simulink model "DualStreamSSR"  (R2021a)
(part 4 of 5)

      KernelAllAttrs=|
      | s[12;12;9;9;19;14;21;23;24;21;12;24;26;26;26;27;28;9;21;23;23;23;24;25;14;19;19;29]@FunctionNameDeclFileNamePortNamesPortTypesPortSerializedTypesPortDirectionsPortWindowSizeEnablesPortWindowMarginEnablesPortSynchronicityEnablesPortSignalSizeEnablesFunctionDeclFunctionTemplateSpecKindFunctionTemplateParamNamesFunctionTemplateParamKindsFunctionTemplateParamTypesFunctionTemplateParamValuesFunctionTemplateParamEnablesClassDeclClassTemplateSpecKindClassTemplateParamNamesClassTemplateParamKindsClassTemplateParamTypesClassTemplateParamValuesClassTemplateParamEnablesClassCtorDeclsClassCtorParamNamesClassCtorParamTypesClassCtorParamSerializedTypes[1 1]@C[28 1]@t6@filtert42@../../../aie/aie_kernels/FirDoubleStream.hC[4 1]@t4@sin1t4@sin2t3@cint4@coutC[4 1]@t30@input_stream_cint16 * restrictt30@input_stream_cint16 * restrictt26@input_stream< cacc48_t > *t27@output_stream< cacc48_t > *C[4 1]@t37@{Q2{P{Tinput_stream{1{t{Scint16}}}}}}t37@{Q2{P{Tinput_stream{1{t{Scint16}}}}}}t35@{P{Tinput_stream{1{t{Scacc48_t}}}}}t36@{P{Toutput_stream{1{t{Scacc48_t}}}}}C[4 1]@t5@inputt5@inputt5@inputt6@outputC[4 1]@l0@l0@l0@l0@C[4 1]@l0@l0@l0@l0@C[4 1]@l0@l0@l0@l0@C[4 1]@l0@l0@l0@l1@t281@namespace DoubleStream {
      | template < int NSamples, int ShiftAcc, bool DiscardSample, bool SwapRead > 
      | void FIR_MultiKernel_cincout::
      | filter(input_stream_cint16 * restrict sin1, input_stream_cint16 * restrict sin2, input_stream< cacc48_t > * cin, output_stream< cacc48_t > * cout);
      | }t4@nonee[0 1]@e[0 1]@e[0 1]@e[0 1]@e[0 1]@t132@namespace DoubleStream {
      | template < int NSamples, int ShiftAcc, bool DiscardSample, bool SwapRead > class FIR_MultiKernel_cincout;
      | }t8@implicitC[4 1]@t8@NSamplest8@ShiftAcct13@DiscardSamplet8@SwapReadC[4 1]@t7@nontypet7@nontypet7@nontypet7@nontypeC[4 1]@t3@intt3@intt4@boolt4@boolC[4 1]@nnnnC[4 1]@l1@l1@l1@l1@C[1 1]@t54@FIR_MultiKernel_cincout(cint16 const ( & taps ) [ 4 ])C[1 1]@C[1 1]@t4@tapsC[1 1]@C[1 1]@t23@cint16 const ( &) [ 4 ]C[1 1]@C[1 1]@t20@{R{Q1{C{Scint16}4}}}
      FunctionDecl=|
      | namespace DoubleStream {
      | template < int NSamples, int ShiftAcc, bool DiscardSample, bool SwapRead > 
      | void FIR_MultiKernel_cincout::
      | filter(input_stream_cint16 * restrict sin1, input_stream_cint16 * restrict sin2, input_stream< cacc48_t > * cin, output_stream< cacc48_t > * cout);
      | }
      ClassDeclTypeOptions=|
      | C[1 1]@t132@namespace DoubleStream {
      | template < int NSamples, int ShiftAcc, bool DiscardSample, bool SwapRead > class FIR_MultiKernel_cincout;
      | }
      ClassDecl=|
      | namespace DoubleStream {
      | template < int NSamples, int ShiftAcc, bool DiscardSample, bool SwapRead > class FIR_MultiKernel_cincout;
      | }
  filter53 : aieBasic/AIE Class Kernel  KernelAllAttrs=|  PortNames={'sin1'; 'sin2'; 'cin'; 'cout'}  PortSerializedTypes={'{Q2{P{Tinput_stream{1{t{Scint16}}}}}}'; '{Q2{P{Tinput_stream{1{t{Scint16}}}}}}'; '{P{Tinput_stream{1{t{Scacc48_t}}}}}'; '{P{Toutput_stream{1{t{Scacc48_t}}}}}'}  PortWindowSizes={0.000000000000000000e+00; 0.000000000000000000e+00; 0.000000000000000000e+00; 0.000000000000000000e+00}  PortWindowMargins={0.000000000000000000e+00; 0.000000000000000000e+00; 0.000000000000000000e+00; 0.000000000000000000e+00}  PortSynchronicities={'auto'; 'auto'; 'auto'; 'auto'}  PortSignalSizes={0.000000000000000000e+00; 0.000000000000000000e+00; 0.000000000000000000e+00; 8.000000000000000000e+00}  ClassTemplateSpecKind=implicit  ClassTemplateParamNames={'NSamples'; 'ShiftAcc'; 'DiscardSample'; 'SwapRead'}  ClassTemplateParamKinds={'nontype'; 'nontype'; 'nontype'; 'nontype'}  ClassTemplateParamTypes={'int'; 'int'; 'bool'; 'bool'}  ClassTemplateParamValues={'512', '15', '0', '0'}  ClassCtorParamNames={'taps'}  ClassCtorParamSerializedTypes={'{R{Q1{C{Scint16}4}}}'}  ClassCtorParamValues={'[-54-21i 102-525i 8773-2748i 342+439i]'}  ClassIndex=1  ClassCtorIndex=1  ClassTabVisible=on  ClassTemplateParamsVisible=on  ClassCtorDeclVisible=on  ClassCtorParamsVisible=on  FunctionTabVisible=on  FunctionDecl=|  PortAttrs={ 'input', 'sin1', 'input_stream_cint16 * restrict', '', '', '', ''; 'input', 'sin2', 'input_stream_cint16 * restrict', '', '', '', ''; 'input', 'cin', 'input_stream< cacc48_t > *', '', '', '', ''; 'output', 'cout', 'output_stream< cacc48_t > *', '', '', '', 'OUTPUT_SIZE' }  PortAttrsEnables={'off', 'off', 'off', 'off', 'off', 'off', 'off';'off', 'off', 'off', 'off', 'off', 'off', 'off';'off', 'off', 'off', 'off', 'off', 'off', 'off';'off', 'off', 'off', 'off', 'off', 'off', 'on'}  SampleTime=-1  ClassDeclTypeOptions=|  ClassDecl=|  ClassTemplateParams={ 'NSamples', 'int', 'BURST_LENGTH'; 'ShiftAcc', 'int', 'SHIFT_ACC'; 'DiscardSample', 'bool', 'FALSE'; 'SwapRead', 'bool', 'FALSE' }  ClassTemplateParamsEnables={'off', 'off', 'on';'off', 'off', 'on';'off', 'off', 'on';'off', 'off', 'on'}  ClassCtorDeclTypeOptions=C[1 1]@t54@FIR_MultiKernel_cincout(cint16 const ( & taps ) [ 4 ])  ClassCtorDecl=FIR_MultiKernel_cincout(cint16 const ( & taps ) [ 4 ])  ClassCtorParams={ 'taps', 'cint16 const ( &) [ 4 ]', 'phi_0' }  KernelHeaderFile=FirDoubleStream.h  KernelClassName=DoubleStream::FIR_MultiKernel_cincout  KernelFunction=filter  KernelSourceFile=FirDoubleStream.cpp  KernelSearchPaths={'$SRC/aie_kernels'}  PreProcOptions={}  CoreRuntimeRatio=0.9  KernelLocSpec=off  ColRowLocation=[0 0]  blockJsonConstraints="{\"type\":\"constraint\",\"constraintType\":\"coreUtilization\",\"sid\":\"838\",\"lhs\":{\"type\":\"runtimeRatio\",\"args\":{\"type\":\"kernel\",\"name\":\"DualStreamSSR_b/Subsystem/filter53\",\"sid\":\"838\"}},\"rhs\":{\"type\":\"evaluable\",\"expr\":\"0.9\",\"value\":0.9},\"equality\":true}"  deprecateConstraints=1
      KernelAllAttrs=|
      | s[12;12;9;9;19;14;21;23;24;21;12;24;26;26;26;27;28;9;21;23;23;23;24;25;14;19;19;29]@FunctionNameDeclFileNamePortNamesPortTypesPortSerializedTypesPortDirectionsPortWindowSizeEnablesPortWindowMarginEnablesPortSynchronicityEnablesPortSignalSizeEnablesFunctionDeclFunctionTemplateSpecKindFunctionTemplateParamNamesFunctionTemplateParamKindsFunctionTemplateParamTypesFunctionTemplateParamValuesFunctionTemplateParamEnablesClassDeclClassTemplateSpecKindClassTemplateParamNamesClassTemplateParamKindsClassTemplateParamTypesClassTemplateParamValuesClassTemplateParamEnablesClassCtorDeclsClassCtorParamNamesClassCtorParamTypesClassCtorParamSerializedTypes[1 1]@C[28 1]@t6@filtert42@../../../aie/aie_kernels/FirDoubleStream.hC[4 1]@t4@sin1t4@sin2t3@cint4@coutC[4 1]@t30@input_stream_cint16 * restrictt30@input_stream_cint16 * restrictt26@input_stream< cacc48_t > *t27@output_stream< cacc48_t > *C[4 1]@t37@{Q2{P{Tinput_stream{1{t{Scint16}}}}}}t37@{Q2{P{Tinput_stream{1{t{Scint16}}}}}}t35@{P{Tinput_stream{1{t{Scacc48_t}}}}}t36@{P{Toutput_stream{1{t{Scacc48_t}}}}}C[4 1]@t5@inputt5@inputt5@inputt6@outputC[4 1]@l0@l0@l0@l0@C[4 1]@l0@l0@l0@l0@C[4 1]@l0@l0@l0@l0@C[4 1]@l0@l0@l0@l1@t281@namespace DoubleStream {
      | template < int NSamples, int ShiftAcc, bool DiscardSample, bool SwapRead > 
      | void FIR_MultiKernel_cincout::
      | filter(input_stream_cint16 * restrict sin1, input_stream_cint16 * restrict sin2, input_stream< cacc48_t > * cin, output_stream< cacc48_t > * cout);
      | }t4@nonee[0 1]@e[0 1]@e[0 1]@e[0 1]@e[0 1]@t132@namespace DoubleStream {
      | template < int NSamples, int ShiftAcc, bool DiscardSample, bool SwapRead > class FIR_MultiKernel_cincout;
      | }t8@implicitC[4 1]@t8@NSamplest8@ShiftAcct13@DiscardSamplet8@SwapReadC[4 1]@t7@nontypet7@nontypet7@nontypet7@nontypeC[4 1]@t3@intt3@intt4@boolt4@boolC[4 1]@nnnnC[4 1]@l1@l1@l1@l1@C[1 1]@t54@FIR_MultiKernel_cincout(cint16 const ( & taps ) [ 4 ])C[1 1]@C[1 1]@t4@tapsC[1 1]@C[1 1]@t23@cint16 const ( &) [ 4 ]C[1 1]@C[1 1]@t20@{R{Q1{C{Scint16}4}}}
      FunctionDecl=|
      | namespace DoubleStream {
      | template < int NSamples, int ShiftAcc, bool DiscardSample, bool SwapRead > 
      | void FIR_MultiKernel_cincout::
      | filter(input_stream_cint16 * restrict sin1, input_stream_cint16 * restrict sin2, input_stream< cacc48_t > * cin, output_stream< cacc48_t > * cout);
      | }
      ClassDeclTypeOptions=|
      | C[1 1]@t132@namespace DoubleStream {
      | template < int NSamples, int ShiftAcc, bool DiscardSample, bool SwapRead > class FIR_MultiKernel_cincout;
      | }
      ClassDecl=|
      | namespace DoubleStream {
      | template < int NSamples, int ShiftAcc, bool DiscardSample, bool SwapRead > class FIR_MultiKernel_cincout;
      | }
  filter54 : aieBasic/AIE Class Kernel  KernelAllAttrs=|  PortNames={'sin1'; 'sin2'; 'cin'; 'sout1'; 'sout2'}  PortSerializedTypes={'{Q2{P{Tinput_stream{1{t{Scint16}}}}}}'; '{Q2{P{Tinput_stream{1{t{Scint16}}}}}}'; '{P{Tinput_stream{1{t{Scacc48_t}}}}}'; '{Q2{P{Toutput_stream{1{t{Scint16}}}}}}'; '{Q2{P{Toutput_stream{1{t{Scint16}}}}}}'}  PortWindowSizes={0.000000000000000000e+00; 0.000000000000000000e+00; 0.000000000000000000e+00; 0.000000000000000000e+00; 0.000000000000000000e+00}  PortWindowMargins={0.000000000000000000e+00; 0.000000000000000000e+00; 0.000000000000000000e+00; 0.000000000000000000e+00; 0.000000000000000000e+00}  PortSynchronicities={'auto'; 'auto'; 'auto'; 'auto'; 'auto'}  PortSignalSizes={0.000000000000000000e+00; 0.000000000000000000e+00; 0.000000000000000000e+00; 4.000000000000000000e+00; 4.000000000000000000e+00}  ClassTemplateSpecKind=implicit  ClassTemplateParamNames={'NSamples'; 'ShiftAcc'; 'DiscardSample'; 'SwapRead'}  ClassTemplateParamKinds={'nontype'; 'nontype'; 'nontype'; 'nontype'}  ClassTemplateParamTypes={'int'; 'int'; 'bool'; 'bool'}  ClassTemplateParamValues={'512', '15', '0', '0'}  ClassCtorParamNames={'taps'}  ClassCtorParamSerializedTypes={'{R{Q1{C{Scint16}4}}}'}  ClassCtorParamValues={'[-83+21i 237+54i 4086-5221i 146+91i]'}  ClassIndex=1  ClassCtorIndex=1  ClassTabVisible=on  ClassTemplateParamsVisible=on  ClassCtorDeclVisible=on  ClassCtorParamsVisible=on  FunctionTabVisible=on  FunctionDecl=|  PortAttrs={ 'input', 'sin1', 'input_stream_cint16 * restrict', '', '', '', ''; 'input', 'sin2', 'input_stream_cint16 * restrict', '', '', '', ''; 'input', 'cin', 'input_stream< cacc48_t > *', '', '', '', ''; 'output', 'sout1', 'output_stream_cint16 * restrict', '', '', '', 'OUTPUT_SIZE/2'; 'output', 'sout2', 'output_stream_cint16 * restrict', '', '', '', 'OUTPUT_SIZE/2' }  PortAttrsEnables={'off', 'off', 'off', 'off', 'off', 'off', 'off';'off', 'off', 'off', 'off', 'off', 'off', 'off';'off', 'off', 'off', 'off', 'off', 'off', 'off';'off', 'off', 'off', 'off', 'off', 'off', 'on';'off', 'off', 'off', 'off', 'off', 'off', 'on'}  SampleTime=-1  ClassDeclTypeOptions=|  ClassDecl=|  ClassTemplateParams={ 'NSamples', 'int', 'BURST_LENGTH'; 'ShiftAcc', 'int', 'SHIFT_ACC'; 'DiscardSample', 'bool', 'FALSE'; 'SwapRead', 'bool', 'FALSE' }  ClassTemplateParamsEnables={'off', 'off', 'on';'off', 'off', 'on';'off', 'off', 'on';'off', 'off', 'on'}  ClassCtorDeclTypeOptions=C[1 1]@t50@FIR_MultiKernel_cin(cint16 const ( & taps ) [ 4 ])  ClassCtorDecl=FIR_MultiKernel_cin(cint16 const ( & taps ) [ 4 ])  ClassCtorParams={ 'taps', 'cint16 const ( &) [ 4 ]', 'phi_1' }  KernelHeaderFile=FirDoubleStream.h  KernelClassName=DoubleStream::FIR_MultiKernel_cin  KernelFunction=filter  KernelSourceFile=FirDoubleStream.cpp  KernelSearchPaths={'$SRC/aie_kernels'}  PreProcOptions={}  CoreRuntimeRatio=0.9  KernelLocSpec=off  ColRowLocation=[0 0]  blockJsonConstraints="{\"type\":\"constraint\",\"constraintType\":\"coreUtilization\",\"sid\":\"839\",\"lhs\":{\"type\":\"runtimeRatio\",\"args\":{\"type\":\"kernel\",\"name\":\"DualStreamSSR_b/Subsystem/filter54\",\"sid\":\"839\"}},\"rhs\":{\"type\":\"evaluable\",\"expr\":\"0.9\",\"value\":0.9},\"equality\":true}"  deprecateConstraints=1
      KernelAllAttrs=|
      | s[12;12;9;9;19;14;21;23;24;21;12;24;26;26;26;27;28;9;21;23;23;23;24;25;14;19;19;29]@FunctionNameDeclFileNamePortNamesPortTypesPortSerializedTypesPortDirectionsPortWindowSizeEnablesPortWindowMarginEnablesPortSynchronicityEnablesPortSignalSizeEnablesFunctionDeclFunctionTemplateSpecKindFunctionTemplateParamNamesFunctionTemplateParamKindsFunctionTemplateParamTypesFunctionTemplateParamValuesFunctionTemplateParamEnablesClassDeclClassTemplateSpecKindClassTemplateParamNamesClassTemplateParamKindsClassTemplateParamTypesClassTemplateParamValuesClassTemplateParamEnablesClassCtorDeclsClassCtorParamNamesClassCtorParamTypesClassCtorParamSerializedTypes[1 1]@C[28 1]@t6@filtert42@../../../aie/aie_kernels/FirDoubleStream.hC[5 1]@t4@sin1t4@sin2t3@cint5@sout1t5@sout2C[5 1]@t30@input_stream_cint16 * restrictt30@input_stream_cint16 * restrictt26@input_stream< cacc48_t > *t31@output_stream_cint16 * restrictt31@output_stream_cint16 * restrictC[5 1]@t37@{Q2{P{Tinput_stream{1{t{Scint16}}}}}}t37@{Q2{P{Tinput_stream{1{t{Scint16}}}}}}t35@{P{Tinput_stream{1{t{Scacc48_t}}}}}t38@{Q2{P{Toutput_stream{1{t{Scint16}}}}}}t38@{Q2{P{Toutput_stream{1{t{Scint16}}}}}}C[5 1]@t5@inputt5@inputt5@inputt6@outputt6@outputC[5 1]@l0@l0@l0@l0@l0@C[5 1]@l0@l0@l0@l0@l0@C[5 1]@l0@l0@l0@l0@l0@C[5 1]@l0@l0@l0@l1@l1@t321@namespace DoubleStream {
      | template < int NSamples, int ShiftAcc, bool DiscardSample, bool SwapRead > 
      | void FIR_MultiKernel_cin::
      | filter(input_stream_cint16 * restrict sin1, input_stream_cint16 * restrict sin2, input_stream< cacc48_t > * cin, output_stream_cint16 * restrict sout1, output_stream_cint16 * restrict sout2);
      | }t4@nonee[0 1]@e[0 1]@e[0 1]@e[0 1]@e[0 1]@t128@namespace DoubleStream {
      | template < int NSamples, int ShiftAcc, bool DiscardSample, bool SwapRead > class FIR_MultiKernel_cin;
      | }t8@implicitC[4 1]@t8@NSamplest8@ShiftAcct13@DiscardSamplet8@SwapReadC[4 1]@t7@nontypet7@nontypet7@nontypet7@nontypeC[4 1]@t3@intt3@intt4@boolt4@boolC[4 1]@nnnnC[4 1]@l1@l1@l1@l1@C[1 1]@t50@FIR_MultiKernel_cin(cint16 const ( & taps ) [ 4 ])C[1 1]@C[1 1]@t4@tapsC[1 1]@C[1 1]@t23@cint16 const ( &) [ 4 ]C[1 1]@C[1 1]@t20@{R{Q1{C{Scint16}4}}}
      FunctionDecl=|
      | namespace DoubleStream {
      | template < int NSamples, int ShiftAcc, bool DiscardSample, bool SwapRead > 
      | void FIR_MultiKernel_cin::
      | filter(input_stream_cint16 * restrict sin1, input_stream_cint16 * restrict sin2, input_stream< cacc48_t > * cin, output_stream_cint16 * restrict sout1, output_stream_cint16 * restrict sout2);
      | }
      ClassDeclTypeOptions=|
      | C[1 1]@t128@namespace DoubleStream {
      | template < int NSamples, int ShiftAcc, bool DiscardSample, bool SwapRead > class FIR_MultiKernel_cin;
      | }
      ClassDecl=|
      | namespace DoubleStream {
      | template < int NSamples, int ShiftAcc, bool DiscardSample, bool SwapRead > class FIR_MultiKernel_cin;
      | }
  filter55 : aieBasic/AIE Class Kernel  KernelAllAttrs=|  PortNames={'sin1'; 'sin2'; 'cin'; 'cout'}  PortSerializedTypes={'{Q2{P{Tinput_stream{1{t{Scint16}}}}}}'; '{Q2{P{Tinput_stream{1{t{Scint16}}}}}}'; '{P{Tinput_stream{1{t{Scacc48_t}}}}}'; '{P{Toutput_stream{1{t{Scacc48_t}}}}}'}  PortWindowSizes={0.000000000000000000e+00; 0.000000000000000000e+00; 0.000000000000000000e+00; 0.000000000000000000e+00}  PortWindowMargins={0.000000000000000000e+00; 0.000000000000000000e+00; 0.000000000000000000e+00; 0.000000000000000000e+00}  PortSynchronicities={'auto'; 'auto'; 'auto'; 'auto'}  PortSignalSizes={0.000000000000000000e+00; 0.000000000000000000e+00; 0.000000000000000000e+00; 8.000000000000000000e+00}  ClassTemplateSpecKind=implicit  ClassTemplateParamNames={'NSamples'; 'ShiftAcc'; 'DiscardSample'; 'SwapRead'}  ClassTemplateParamKinds={'nontype'; 'nontype'; 'nontype'; 'nontype'}  ClassTemplateParamTypes={'int'; 'int'; 'bool'; 'bool'}  ClassTemplateParamValues={'512', '15', '1', '0'}  ClassCtorParamNames={'taps'}  ClassCtorParamSerializedTypes={'{R{Q1{C{Scint16}4}}}'}  ClassCtorParamValues={'[342-439i 8773+2748i 102+525i -54+21i]'}  ClassIndex=1  ClassCtorIndex=1  ClassTabVisible=on  ClassTemplateParamsVisible=on  ClassCtorDeclVisible=on  ClassCtorParamsVisible=on  FunctionTabVisible=on  FunctionDecl=|  PortAttrs={ 'input', 'sin1', 'input_stream_cint16 * restrict', '', '', '', ''; 'input', 'sin2', 'input_stream_cint16 * restrict', '', '', '', ''; 'input', 'cin', 'input_stream< cacc48_t > *', '', '', '', ''; 'output', 'cout', 'output_stream< cacc48_t > *', '', '', '', 'OUTPUT_SIZE' }  PortAttrsEnables={'off', 'off', 'off', 'off', 'off', 'off', 'off';'off', 'off', 'off', 'off', 'off', 'off', 'off';'off', 'off', 'off', 'off', 'off', 'off', 'off';'off', 'off', 'off', 'off', 'off', 'off', 'on'}  SampleTime=-1  ClassDeclTypeOptions=|  ClassDecl=|  ClassTemplateParams={ 'NSamples', 'int', 'BURST_LENGTH'; 'ShiftAcc', 'int', 'SHIFT_ACC'; 'DiscardSample', 'bool', 'TRUE'; 'SwapRead', 'bool', 'FALSE' }  ClassTemplateParamsEnables={'off', 'off', 'on';'off', 'off', 'on';'off', 'off', 'on';'off', 'off', 'on'}  ClassCtorDeclTypeOptions=C[1 1]@t54@FIR_MultiKernel_cincout(cint16 const ( & taps ) [ 4 ])  ClassCtorDecl=FIR_MultiKernel_cincout(cint16 const ( & taps ) [ 4 ])  ClassCtorParams={ 'taps', 'cint16 const ( &) [ 4 ]', 'phi_7' }  KernelHeaderFile=FirDoubleStream.h  KernelClassName=DoubleStream::FIR_MultiKernel_cincout  KernelFunction=filter  KernelSourceFile=FirDoubleStream.cpp  KernelSearchPaths={'$SRC/aie_kernels'}  PreProcOptions={}  CoreRuntimeRatio=0.9  KernelLocSpec=off  ColRowLocation=[0 0]  blockJsonConstraints="{\"type\":\"constraint\",\"constraintType\":\"coreUtilization\",\"sid\":\"840\",\"lhs\":{\"type\":\"runtimeRatio\",\"args\":{\"type\":\"kernel\",\"name\":\"DualStreamSSR_b/Subsystem/filter55\",\"sid\":\"840\"}},\"rhs\":{\"type\":\"evaluable\",\"expr\":\"0.9\",\"value\":0.9},\"equality\":true}"  deprecateConstraints=1
      KernelAllAttrs=|
      | s[12;12;9;9;19;14;21;23;24;21;12;24;26;26;26;27;28;9;21;23;23;23;24;25;14;19;19;29]@FunctionNameDeclFileNamePortNamesPortTypesPortSerializedTypesPortDirectionsPortWindowSizeEnablesPortWindowMarginEnablesPortSynchronicityEnablesPortSignalSizeEnablesFunctionDeclFunctionTemplateSpecKindFunctionTemplateParamNamesFunctionTemplateParamKindsFunctionTemplateParamTypesFunctionTemplateParamValuesFunctionTemplateParamEnablesClassDeclClassTemplateSpecKindClassTemplateParamNamesClassTemplateParamKindsClassTemplateParamTypesClassTemplateParamValuesClassTemplateParamEnablesClassCtorDeclsClassCtorParamNamesClassCtorParamTypesClassCtorParamSerializedTypes[1 1]@C[28 1]@t6@filtert42@../../../aie/aie_kernels/FirDoubleStream.hC[4 1]@t4@sin1t4@sin2t3@cint4@coutC[4 1]@t30@input_stream_cint16 * restrictt30@input_stream_cint16 * restrictt26@input_stream< cacc48_t > *t27@output_stream< cacc48_t > *C[4 1]@t37@{Q2{P{Tinput_stream{1{t{Scint16}}}}}}t37@{Q2{P{Tinput_stream{1{t{Scint16}}}}}}t35@{P{Tinput_stream{1{t{Scacc48_t}}}}}t36@{P{Toutput_stream{1{t{Scacc48_t}}}}}C[4 1]@t5@inputt5@inputt5@inputt6@outputC[4 1]@l0@l0@l0@l0@C[4 1]@l0@l0@l0@l0@C[4 1]@l0@l0@l0@l0@C[4 1]@l0@l0@l0@l1@t281@namespace DoubleStream {
      | template < int NSamples, int ShiftAcc, bool DiscardSample, bool SwapRead > 
      | void FIR_MultiKernel_cincout::
      | filter(input_stream_cint16 * restrict sin1, input_stream_cint16 * restrict sin2, input_stream< cacc48_t > * cin, output_stream< cacc48_t > * cout);
      | }t4@nonee[0 1]@e[0 1]@e[0 1]@e[0 1]@e[0 1]@t132@namespace DoubleStream {
      | template < int NSamples, int ShiftAcc, bool DiscardSample, bool SwapRead > class FIR_MultiKernel_cincout;
      | }t8@implicitC[4 1]@t8@NSamplest8@ShiftAcct13@DiscardSamplet8@SwapReadC[4 1]@t7@nontypet7@nontypet7@nontypet7@nontypeC[4 1]@t3@intt3@intt4@boolt4@boolC[4 1]@nnnnC[4 1]@l1@l1@l1@l1@C[1 1]@t54@FIR_MultiKernel_cincout(cint16 const ( & taps ) [ 4 ])C[1 1]@C[1 1]@t4@tapsC[1 1]@C[1 1]@t23@cint16 const ( &) [ 4 ]C[1 1]@C[1 1]@t20@{R{Q1{C{Scint16}4}}}
      FunctionDecl=|
      | namespace DoubleStream {
      | template < int NSamples, int ShiftAcc, bool DiscardSample, bool SwapRead > 
      | void FIR_MultiKernel_cincout::
      | filter(input_stream_cint16 * restrict sin1, input_stream_cint16 * restrict sin2, input_stream< cacc48_t > * cin, output_stream< cacc48_t > * cout);
      | }
      ClassDeclTypeOptions=|
      | C[1 1]@t132@namespace DoubleStream {
      | template < int NSamples, int ShiftAcc, bool DiscardSample, bool SwapRead > class FIR_MultiKernel_cincout;
      | }
      ClassDecl=|
      | namespace DoubleStream {
      | template < int NSamples, int ShiftAcc, bool DiscardSample, bool SwapRead > class FIR_MultiKernel_cincout;
      | }
  filter56 : aieBasic/AIE Class Kernel  KernelAllAttrs=|  PortNames={'sin1'; 'sin2'; 'cout'}  PortSerializedTypes={'{Q2{P{Tinput_stream{1{t{Scint16}}}}}}'; '{Q2{P{Tinput_stream{1{t{Scint16}}}}}}'; '{P{Toutput_stream{1{t{Scacc48_t}}}}}'}  PortWindowSizes={0.000000000000000000e+00; 0.000000000000000000e+00; 0.000000000000000000e+00}  PortWindowMargins={0.000000000000000000e+00; 0.000000000000000000e+00; 0.000000000000000000e+00}  PortSynchronicities={'auto'; 'auto'; 'auto'}  PortSignalSizes={0.000000000000000000e+00; 0.000000000000000000e+00; 8.000000000000000000e+00}  ClassTemplateSpecKind=implicit  ClassTemplateParamNames={'NSamples'; 'ShiftAcc'; 'DiscardSample'; 'SwapRead'}  ClassTemplateParamKinds={'nontype'; 'nontype'; 'nontype'; 'nontype'}  ClassTemplateParamTypes={'int'; 'int'; 'bool'; 'bool'}  ClassTemplateParamValues={'512', '15', '0', '0'}  ClassCtorParamNames={'taps'}  ClassCtorParamSerializedTypes={'{R{Q1{C{Scint16}4}}}'}  ClassCtorParamValues={'[-54-21i 102-525i 8773-2748i 342+439i]'}  ClassIndex=1  ClassCtorIndex=1  ClassTabVisible=on  ClassTemplateParamsVisible=on  ClassCtorDeclVisible=on  ClassCtorParamsVisible=on  FunctionTabVisible=on  FunctionDecl=|  PortAttrs={ 'input', 'sin1', 'input_stream_cint16 * restrict', '', '', '', ''; 'input', 'sin2', 'input_stream_cint16 * restrict', '', '', '', ''; 'output', 'cout', 'output_stream< cacc48_t > *', '', '', '', 'OUTPUT_SIZE' }  PortAttrsEnables={'off', 'off', 'off', 'off', 'off', 'off', 'off';'off', 'off', 'off', 'off', 'off', 'off', 'off';'off', 'off', 'off', 'off', 'off', 'off', 'on'}  SampleTime=-1  ClassDeclTypeOptions=|  ClassDecl=|  ClassTemplateParams={ 'NSamples', 'int', 'BURST_LENGTH'; 'ShiftAcc', 'int', 'SHIFT_ACC'; 'DiscardSample', 'bool', 'FALSE'; 'SwapRead', 'bool', 'FALSE' }  ClassTemplateParamsEnables={'off', 'off', 'on';'off', 'off', 'on';'off', 'off', 'on';'off', 'off', 'on'}  ClassCtorDeclTypeOptions=C[1 1]@t51@FIR_MultiKernel_cout(cint16 const ( & taps ) [ 4 ])  ClassCtorDecl=FIR_MultiKernel_cout(cint16 const ( & taps ) [ 4 ])  ClassCtorParams={ 'taps', 'cint16 const ( &) [ 4 ]', 'phi_0' }  KernelHeaderFile=FirDoubleStream.h  KernelClassName=DoubleStream::FIR_MultiKernel_cout  KernelFunction=filter  KernelSourceFile=FirDoubleStream.cpp  KernelSearchPaths={'$SRC/aie_kernels'}  PreProcOptions={}  CoreRuntimeRatio=0.9  KernelLocSpec=off  ColRowLocation=[0 0]  blockJsonConstraints="[{\"type\":\"constraint\",\"constraintType\":\"coreUtilization\",\"sid\":\"841\",\"lhs\":{\"type\":\"runtimeRatio\",\"args\":{\"type\":\"kernel\",\"name\":\"DualStreamSSR/SSR8/filter56\",\"sid\":\"841\"}},\"rhs\":{\"type\":\"evaluable\",\"expr\":\"0.9\",\"value\":0.9},\"equality\":true},{\"type\":\"constraint\",\"constraintType\":\"location_kernel\",\"sid\":\"841\",\"lhs\":{\"type\":\"location\",\"templParam\":\"kernel\",\"args\":{\"type\":\"kernel\",\"name\":\"DualStreamSSR/SSR8/filter56\",\"sid\":\"841\"}},\"rhs\":{\"type\":\"tile\",\"args\":[{\"type\":\"evaluable\",\"expr\":\"30\",\"value\":30},{\"type\":\"evaluable\",\"expr\":\"7\",\"value\":7}]},\"equality\":true}]"  deprecateConstraints=1
      KernelAllAttrs=|
      | s[12;12;9;9;19;14;21;23;24;21;12;24;26;26;26;27;28;9;21;23;23;23;24;25;14;19;19;29]@FunctionNameDeclFileNamePortNamesPortTypesPortSerializedTypesPortDirectionsPortWindowSizeEnablesPortWindowMarginEnablesPortSynchronicityEnablesPortSignalSizeEnablesFunctionDeclFunctionTemplateSpecKindFunctionTemplateParamNamesFunctionTemplateParamKindsFunctionTemplateParamTypesFunctionTemplateParamValuesFunctionTemplateParamEnablesClassDeclClassTemplateSpecKindClassTemplateParamNamesClassTemplateParamKindsClassTemplateParamTypesClassTemplateParamValuesClassTemplateParamEnablesClassCtorDeclsClassCtorParamNamesClassCtorParamTypesClassCtorParamSerializedTypes[1 1]@C[28 1]@t6@filtert42@../../../aie/aie_kernels/FirDoubleStream.hC[3 1]@t4@sin1t4@sin2t4@coutC[3 1]@t30@input_stream_cint16 * restrictt30@input_stream_cint16 * restrictt27@output_stream< cacc48_t > *C[3 1]@t37@{Q2{P{Tinput_stream{1{t{Scint16}}}}}}t37@{Q2{P{Tinput_stream{1{t{Scint16}}}}}}t36@{P{Toutput_stream{1{t{Scacc48_t}}}}}C[3 1]@t5@inputt5@inputt6@outputC[3 1]@l0@l0@l0@C[3 1]@l0@l0@l0@C[3 1]@l0@l0@l0@C[3 1]@l0@l0@l1@t246@namespace DoubleStream {
      | template < int NSamples, int ShiftAcc, bool DiscardSample, bool SwapRead > 
      | void FIR_MultiKernel_cout::
      | filter(input_stream_cint16 * restrict sin1, input_stream_cint16 * restrict sin2, output_stream< cacc48_t > * cout);
      | }t4@nonee[0 1]@e[0 1]@e[0 1]@e[0 1]@e[0 1]@t129@namespace DoubleStream {
      | template < int NSamples, int ShiftAcc, bool DiscardSample, bool SwapRead > class FIR_MultiKernel_cout;
      | }t8@implicitC[4 1]@t8@NSamplest8@ShiftAcct13@DiscardSamplet8@SwapReadC[4 1]@t7@nontypet7@nontypet7@nontypet7@nontypeC[4 1]@t3@intt3@intt4@boolt4@boolC[4 1]@nnnnC[4 1]@l1@l1@l1@l1@C[1 1]@t51@FIR_MultiKernel_cout(cint16 const ( & taps ) [ 4 ])C[1 1]@C[1 1]@t4@tapsC[1 1]@C[1 1]@t23@cint16 const ( &) [ 4 ]C[1 1]@C[1 1]@t20@{R{Q1{C{Scint16}4}}}
      FunctionDecl=|
      | namespace DoubleStream {
      | template < int NSamples, int ShiftAcc, bool DiscardSample, bool SwapRead > 
      | void FIR_MultiKernel_cout::
      | filter(input_stream_cint16 * restrict sin1, input_stream_cint16 * restrict sin2, output_stream< cacc48_t > * cout);
      | }
      ClassDeclTypeOptions=|
      | C[1 1]@t129@namespace DoubleStream {
      | template < int NSamples, int ShiftAcc, bool DiscardSample, bool SwapRead > class FIR_MultiKernel_cout;
      | }
      ClassDecl=|
      | namespace DoubleStream {
      | template < int NSamples, int ShiftAcc, bool DiscardSample, bool SwapRead > class FIR_MultiKernel_cout;
      | }
  filter57 : aieBasic/AIE Class Kernel  KernelAllAttrs=|  PortNames={'sin1'; 'sin2'; 'cin'; 'cout'}  PortSerializedTypes={'{Q2{P{Tinput_stream{1{t{Scint16}}}}}}'; '{Q2{P{Tinput_stream{1{t{Scint16}}}}}}'; '{P{Tinput_stream{1{t{Scacc48_t}}}}}'; '{P{Toutput_stream{1{t{Scacc48_t}}}}}'}  PortWindowSizes={0.000000000000000000e+00; 0.000000000000000000e+00; 0.000000000000000000e+00; 0.000000000000000000e+00}  PortWindowMargins={0.000000000000000000e+00; 0.000000000000000000e+00; 0.000000000000000000e+00; 0.000000000000000000e+00}  PortSynchronicities={'auto'; 'auto'; 'auto'; 'auto'}  PortSignalSizes={0.000000000000000000e+00; 0.000000000000000000e+00; 0.000000000000000000e+00; 8.000000000000000000e+00}  ClassTemplateSpecKind=implicit  ClassTemplateParamNames={'NSamples'; 'ShiftAcc'; 'DiscardSample'; 'SwapRead'}  ClassTemplateParamKinds={'nontype'; 'nontype'; 'nontype'; 'nontype'}  ClassTemplateParamTypes={'int'; 'int'; 'bool'; 'bool'}  ClassTemplateParamValues={'512', '15', '1', '0'}  ClassCtorParamNames={'taps'}  ClassCtorParamSerializedTypes={'{R{Q1{C{Scint16}4}}}'}  ClassCtorParamValues={'[342-439i 8773+2748i 102+525i -54+21i]'}  ClassIndex=1  ClassCtorIndex=1  ClassTabVisible=on  ClassTemplateParamsVisible=on  ClassCtorDeclVisible=on  ClassCtorParamsVisible=on  FunctionTabVisible=on  FunctionDecl=|  PortAttrs={ 'input', 'sin1', 'input_stream_cint16 * restrict', '', '', '', ''; 'input', 'sin2', 'input_stream_cint16 * restrict', '', '', '', ''; 'input', 'cin', 'input_stream< cacc48_t > *', '', '', '', ''; 'output', 'cout', 'output_stream< cacc48_t > *', '', '', '', 'OUTPUT_SIZE' }  PortAttrsEnables={'off', 'off', 'off', 'off', 'off', 'off', 'off';'off', 'off', 'off', 'off', 'off', 'off', 'off';'off', 'off', 'off', 'off', 'off', 'off', 'off';'off', 'off', 'off', 'off', 'off', 'off', 'on'}  SampleTime=-1  ClassDeclTypeOptions=|  ClassDecl=|  ClassTemplateParams={ 'NSamples', 'int', 'BURST_LENGTH'; 'ShiftAcc', 'int', 'SHIFT_ACC'; 'DiscardSample', 'bool', 'TRUE'; 'SwapRead', 'bool', 'FALSE' }  ClassTemplateParamsEnables={'off', 'off', 'on';'off', 'off', 'on';'off', 'off', 'on';'off', 'off', 'on'}  ClassCtorDeclTypeOptions=C[1 1]@t54@FIR_MultiKernel_cincout(cint16 const ( & taps ) [ 4 ])  ClassCtorDecl=FIR_MultiKernel_cincout(cint16 const ( & taps ) [ 4 ])  ClassCtorParams={ 'taps', 'cint16 const ( &) [ 4 ]', 'phi_7' }  KernelHeaderFile=FirDoubleStream.h  KernelClassName=DoubleStream::FIR_MultiKernel_cincout  KernelFunction=filter  KernelSourceFile=FirDoubleStream.cpp  KernelSearchPaths={'$SRC/aie_kernels'}  PreProcOptions={}  CoreRuntimeRatio=0.9  KernelLocSpec=off  ColRowLocation=[0 0]  blockJsonConstraints="{\"type\":\"constraint\",\"constraintType\":\"coreUtilization\",\"sid\":\"842\",\"lhs\":{\"type\":\"runtimeRatio\",\"args\":{\"type\":\"kernel\",\"name\":\"DualStreamSSR_b/Subsystem/filter57\",\"sid\":\"842\"}},\"rhs\":{\"type\":\"evaluable\",\"expr\":\"0.9\",\"value\":0.9},\"equality\":true}"  deprecateConstraints=1
      KernelAllAttrs=|
      | s[12;12;9;9;19;14;21;23;24;21;12;24;26;26;26;27;28;9;21;23;23;23;24;25;14;19;19;29]@FunctionNameDeclFileNamePortNamesPortTypesPortSerializedTypesPortDirectionsPortWindowSizeEnablesPortWindowMarginEnablesPortSynchronicityEnablesPortSignalSizeEnablesFunctionDeclFunctionTemplateSpecKindFunctionTemplateParamNamesFunctionTemplateParamKindsFunctionTemplateParamTypesFunctionTemplateParamValuesFunctionTemplateParamEnablesClassDeclClassTemplateSpecKindClassTemplateParamNamesClassTemplateParamKindsClassTemplateParamTypesClassTemplateParamValuesClassTemplateParamEnablesClassCtorDeclsClassCtorParamNamesClassCtorParamTypesClassCtorParamSerializedTypes[1 1]@C[28 1]@t6@filtert42@../../../aie/aie_kernels/FirDoubleStream.hC[4 1]@t4@sin1t4@sin2t3@cint4@coutC[4 1]@t30@input_stream_cint16 * restrictt30@input_stream_cint16 * restrictt26@input_stream< cacc48_t > *t27@output_stream< cacc48_t > *C[4 1]@t37@{Q2{P{Tinput_stream{1{t{Scint16}}}}}}t37@{Q2{P{Tinput_stream{1{t{Scint16}}}}}}t35@{P{Tinput_stream{1{t{Scacc48_t}}}}}t36@{P{Toutput_stream{1{t{Scacc48_t}}}}}C[4 1]@t5@inputt5@inputt5@inputt6@outputC[4 1]@l0@l0@l0@l0@C[4 1]@l0@l0@l0@l0@C[4 1]@l0@l0@l0@l0@C[4 1]@l0@l0@l0@l1@t281@namespace DoubleStream {
      | template < int NSamples, int ShiftAcc, bool DiscardSample, bool SwapRead > 
      | void FIR_MultiKernel_cincout::
      | filter(input_stream_cint16 * restrict sin1, input_stream_cint16 * restrict sin2, input_stream< cacc48_t > * cin, output_stream< cacc48_t > * cout);
      | }t4@nonee[0 1]@e[0 1]@e[0 1]@e[0 1]@e[0 1]@t132@namespace DoubleStream {
      | template < int NSamples, int ShiftAcc, bool DiscardSample, bool SwapRead > class FIR_MultiKernel_cincout;
      | }t8@implicitC[4 1]@t8@NSamplest8@ShiftAcct13@DiscardSamplet8@SwapReadC[4 1]@t7@nontypet7@nontypet7@nontypet7@nontypeC[4 1]@t3@intt3@intt4@boolt4@boolC[4 1]@nnnnC[4 1]@l1@l1@l1@l1@C[1 1]@t54@FIR_MultiKernel_cincout(cint16 const ( & taps ) [ 4 ])C[1 1]@C[1 1]@t4@tapsC[1 1]@C[1 1]@t23@cint16 const ( &) [ 4 ]C[1 1]@C[1 1]@t20@{R{Q1{C{Scint16}4}}}
      FunctionDecl=|
      | namespace DoubleStream {
      | template < int NSamples, int ShiftAcc, bool DiscardSample, bool SwapRead > 
      | void FIR_MultiKernel_cincout::
      | filter(input_stream_cint16 * restrict sin1, input_stream_cint16 * restrict sin2, input_stream< cacc48_t > * cin, output_stream< cacc48_t > * cout);
      | }
      ClassDeclTypeOptions=|
      | C[1 1]@t132@namespace DoubleStream {
      | template < int NSamples, int ShiftAcc, bool DiscardSample, bool SwapRead > class FIR_MultiKernel_cincout;
      | }
      ClassDecl=|
      | namespace DoubleStream {
      | template < int NSamples, int ShiftAcc, bool DiscardSample, bool SwapRead > class FIR_MultiKernel_cincout;
      | }
  filter58 : aieBasic/AIE Class Kernel  KernelAllAttrs=|  PortNames={'sin1'; 'sin2'; 'cin'; 'cout'}  PortSerializedTypes={'{Q2{P{Tinput_stream{1{t{Scint16}}}}}}'; '{Q2{P{Tinput_stream{1{t{Scint16}}}}}}'; '{P{Tinput_stream{1{t{Scacc48_t}}}}}'; '{P{Toutput_stream{1{t{Scacc48_t}}}}}'}  PortWindowSizes={0.000000000000000000e+00; 0.000000000000000000e+00; 0.000000000000000000e+00; 0.000000000000000000e+00}  PortWindowMargins={0.000000000000000000e+00; 0.000000000000000000e+00; 0.000000000000000000e+00; 0.000000000000000000e+00}  PortSynchronicities={'auto'; 'auto'; 'auto'; 'auto'}  PortSignalSizes={0.000000000000000000e+00; 0.000000000000000000e+00; 0.000000000000000000e+00; 8.000000000000000000e+00}  ClassTemplateSpecKind=implicit  ClassTemplateParamNames={'NSamples'; 'ShiftAcc'; 'DiscardSample'; 'SwapRead'}  ClassTemplateParamKinds={'nontype'; 'nontype'; 'nontype'; 'nontype'}  ClassTemplateParamTypes={'int'; 'int'; 'bool'; 'bool'}  ClassTemplateParamValues={'512', '15', '0', '0'}  ClassCtorParamNames={'taps'}  ClassCtorParamSerializedTypes={'{R{Q1{C{Scint16}4}}}'}  ClassCtorParamValues={'[-54-21i 102-525i 8773-2748i 342+439i]'}  ClassIndex=1  ClassCtorIndex=1  ClassTabVisible=on  ClassTemplateParamsVisible=on  ClassCtorDeclVisible=on  ClassCtorParamsVisible=on  FunctionTabVisible=on  FunctionDecl=|  PortAttrs={ 'input', 'sin1', 'input_stream_cint16 * restrict', '', '', '', ''; 'input', 'sin2', 'input_stream_cint16 * restrict', '', '', '', ''; 'input', 'cin', 'input_stream< cacc48_t > *', '', '', '', ''; 'output', 'cout', 'output_stream< cacc48_t > *', '', '', '', 'OUTPUT_SIZE' }  PortAttrsEnables={'off', 'off', 'off', 'off', 'off', 'off', 'off';'off', 'off', 'off', 'off', 'off', 'off', 'off';'off', 'off', 'off', 'off', 'off', 'off', 'off';'off', 'off', 'off', 'off', 'off', 'off', 'on'}  SampleTime=-1  ClassDeclTypeOptions=|  ClassDecl=|  ClassTemplateParams={ 'NSamples', 'int', 'BURST_LENGTH'; 'ShiftAcc', 'int', 'SHIFT_ACC'; 'DiscardSample', 'bool', 'FALSE'; 'SwapRead', 'bool', 'FALSE' }  ClassTemplateParamsEnables={'off', 'off', 'on';'off', 'off', 'on';'off', 'off', 'on';'off', 'off', 'on'}  ClassCtorDeclTypeOptions=C[1 1]@t54@FIR_MultiKernel_cincout(cint16 const ( & taps ) [ 4 ])  ClassCtorDecl=FIR_MultiKernel_cincout(cint16 const ( & taps ) [ 4 ])  ClassCtorParams={ 'taps', 'cint16 const ( &) [ 4 ]', 'phi_0' }  KernelHeaderFile=FirDoubleStream.h  KernelClassName=DoubleStream::FIR_MultiKernel_cincout  KernelFunction=filter  KernelSourceFile=FirDoubleStream.cpp  KernelSearchPaths={'$SRC/aie_kernels'}  PreProcOptions={}  CoreRuntimeRatio=0.9  KernelLocSpec=off  ColRowLocation=[0 0]  blockJsonConstraints="{\"type\":\"constraint\",\"constraintType\":\"coreUtilization\",\"sid\":\"843\",\"lhs\":{\"type\":\"runtimeRatio\",\"args\":{\"type\":\"kernel\",\"name\":\"DualStreamSSR_b/Subsystem/filter58\",\"sid\":\"843\"}},\"rhs\":{\"type\":\"evaluable\",\"expr\":\"0.9\",\"value\":0.9},\"equality\":true}"  deprecateConstraints=1
      KernelAllAttrs=|
      | s[12;12;9;9;19;14;21;23;24;21;12;24;26;26;26;27;28;9;21;23;23;23;24;25;14;19;19;29]@FunctionNameDeclFileNamePortNamesPortTypesPortSerializedTypesPortDirectionsPortWindowSizeEnablesPortWindowMarginEnablesPortSynchronicityEnablesPortSignalSizeEnablesFunctionDeclFunctionTemplateSpecKindFunctionTemplateParamNamesFunctionTemplateParamKindsFunctionTemplateParamTypesFunctionTemplateParamValuesFunctionTemplateParamEnablesClassDeclClassTemplateSpecKindClassTemplateParamNamesClassTemplateParamKindsClassTemplateParamTypesClassTemplateParamValuesClassTemplateParamEnablesClassCtorDeclsClassCtorParamNamesClassCtorParamTypesClassCtorParamSerializedTypes[1 1]@C[28 1]@t6@filtert42@../../../aie/aie_kernels/FirDoubleStream.hC[4 1]@t4@sin1t4@sin2t3@cint4@coutC[4 1]@t30@input_stream_cint16 * restrictt30@input_stream_cint16 * restrictt26@input_stream< cacc48_t > *t27@output_stream< cacc48_t > *C[4 1]@t37@{Q2{P{Tinput_stream{1{t{Scint16}}}}}}t37@{Q2{P{Tinput_stream{1{t{Scint16}}}}}}t35@{P{Tinput_stream{1{t{Scacc48_t}}}}}t36@{P{Toutput_stream{1{t{Scacc48_t}}}}}C[4 1]@t5@inputt5@inputt5@inputt6@outputC[4 1]@l0@l0@l0@l0@C[4 1]@l0@l0@l0@l0@C[4 1]@l0@l0@l0@l0@C[4 1]@l0@l0@l0@l1@t281@namespace DoubleStream {
      | template < int NSamples, int ShiftAcc, bool DiscardSample, bool SwapRead > 
      | void FIR_MultiKernel_cincout::
      | filter(input_stream_cint16 * restrict sin1, input_stream_cint16 * restrict sin2, input_stream< cacc48_t > * cin, output_stream< cacc48_t > * cout);
      | }t4@nonee[0 1]@e[0 1]@e[0 1]@e[0 1]@e[0 1]@t132@namespace DoubleStream {
      | template < int NSamples, int ShiftAcc, bool DiscardSample, bool SwapRead > class FIR_MultiKernel_cincout;
      | }t8@implicitC[4 1]@t8@NSamplest8@ShiftAcct13@DiscardSamplet8@SwapReadC[4 1]@t7@nontypet7@nontypet7@nontypet7@nontypeC[4 1]@t3@intt3@intt4@boolt4@boolC[4 1]@nnnnC[4 1]@l1@l1@l1@l1@C[1 1]@t54@FIR_MultiKernel_cincout(cint16 const ( & taps ) [ 4 ])C[1 1]@C[1 1]@t4@tapsC[1 1]@C[1 1]@t23@cint16 const ( &) [ 4 ]C[1 1]@C[1 1]@t20@{R{Q1{C{Scint16}4}}}
      FunctionDecl=|
      | namespace DoubleStream {
      | template < int NSamples, int ShiftAcc, bool DiscardSample, bool SwapRead > 
      | void FIR_MultiKernel_cincout::
      | filter(input_stream_cint16 * restrict sin1, input_stream_cint16 * restrict sin2, input_stream< cacc48_t > * cin, output_stream< cacc48_t > * cout);
      | }
      ClassDeclTypeOptions=|
      | C[1 1]@t132@namespace DoubleStream {
      | template < int NSamples, int ShiftAcc, bool DiscardSample, bool SwapRead > class FIR_MultiKernel_cincout;
      | }
      ClassDecl=|
      | namespace DoubleStream {
      | template < int NSamples, int ShiftAcc, bool DiscardSample, bool SwapRead > class FIR_MultiKernel_cincout;
      | }
  filter59 : aieBasic/AIE Class Kernel  KernelAllAttrs=|  PortNames={'sin1'; 'sin2'; 'cin'; 'cout'}  PortSerializedTypes={'{Q2{P{Tinput_stream{1{t{Scint16}}}}}}'; '{Q2{P{Tinput_stream{1{t{Scint16}}}}}}'; '{P{Tinput_stream{1{t{Scacc48_t}}}}}'; '{P{Toutput_stream{1{t{Scacc48_t}}}}}'}  PortWindowSizes={0.000000000000000000e+00; 0.000000000000000000e+00; 0.000000000000000000e+00; 0.000000000000000000e+00}  PortWindowMargins={0.000000000000000000e+00; 0.000000000000000000e+00; 0.000000000000000000e+00; 0.000000000000000000e+00}  PortSynchronicities={'auto'; 'auto'; 'auto'; 'auto'}  PortSignalSizes={0.000000000000000000e+00; 0.000000000000000000e+00; 0.000000000000000000e+00; 8.000000000000000000e+00}  ClassTemplateSpecKind=implicit  ClassTemplateParamNames={'NSamples'; 'ShiftAcc'; 'DiscardSample'; 'SwapRead'}  ClassTemplateParamKinds={'nontype'; 'nontype'; 'nontype'; 'nontype'}  ClassTemplateParamTypes={'int'; 'int'; 'bool'; 'bool'}  ClassTemplateParamValues={'512', '15', '0', '0'}  ClassCtorParamNames={'taps'}  ClassCtorParamSerializedTypes={'{R{Q1{C{Scint16}4}}}'}  ClassCtorParamValues={'[-83+21i 237+54i 4086-5221i 146+91i]'}  ClassIndex=1  ClassCtorIndex=1  ClassTabVisible=on  ClassTemplateParamsVisible=on  ClassCtorDeclVisible=on  ClassCtorParamsVisible=on  FunctionTabVisible=on  FunctionDecl=|  PortAttrs={ 'input', 'sin1', 'input_stream_cint16 * restrict', '', '', '', ''; 'input', 'sin2', 'input_stream_cint16 * restrict', '', '', '', ''; 'input', 'cin', 'input_stream< cacc48_t > *', '', '', '', ''; 'output', 'cout', 'output_stream< cacc48_t > *', '', '', '', 'OUTPUT_SIZE' }  PortAttrsEnables={'off', 'off', 'off', 'off', 'off', 'off', 'off';'off', 'off', 'off', 'off', 'off', 'off', 'off';'off', 'off', 'off', 'off', 'off', 'off', 'off';'off', 'off', 'off', 'off', 'off', 'off', 'on'}  SampleTime=-1  ClassDeclTypeOptions=|  ClassDecl=|  ClassTemplateParams={ 'NSamples', 'int', 'BURST_LENGTH'; 'ShiftAcc', 'int', 'SHIFT_ACC'; 'DiscardSample', 'bool', 'FALSE'; 'SwapRead', 'bool', 'FALSE' }  ClassTemplateParamsEnables={'off', 'off', 'on';'off', 'off', 'on';'off', 'off', 'on';'off', 'off', 'on'}  ClassCtorDeclTypeOptions=C[1 1]@t54@FIR_MultiKernel_cincout(cint16 const ( & taps ) [ 4 ])  ClassCtorDecl=FIR_MultiKernel_cincout(cint16 const ( & taps ) [ 4 ])  ClassCtorParams={ 'taps', 'cint16 const ( &) [ 4 ]', 'phi_1' }  KernelHeaderFile=FirDoubleStream.h  KernelClassName=DoubleStream::FIR_MultiKernel_cincout  KernelFunction=filter  KernelSourceFile=FirDoubleStream.cpp  KernelSearchPaths={'$SRC/aie_kernels'}  PreProcOptions={}  CoreRuntimeRatio=0.9  KernelLocSpec=off  ColRowLocation=[0 0]  blockJsonConstraints="{\"type\":\"constraint\",\"constraintType\":\"coreUtilization\",\"sid\":\"844\",\"lhs\":{\"type\":\"runtimeRatio\",\"args\":{\"type\":\"kernel\",\"name\":\"DualStreamSSR_b/Subsystem/filter59\",\"sid\":\"844\"}},\"rhs\":{\"type\":\"evaluable\",\"expr\":\"0.9\",\"value\":0.9},\"equality\":true}"  deprecateConstraints=1
      KernelAllAttrs=|
      | s[12;12;9;9;19;14;21;23;24;21;12;24;26;26;26;27;28;9;21;23;23;23;24;25;14;19;19;29]@FunctionNameDeclFileNamePortNamesPortTypesPortSerializedTypesPortDirectionsPortWindowSizeEnablesPortWindowMarginEnablesPortSynchronicityEnablesPortSignalSizeEnablesFunctionDeclFunctionTemplateSpecKindFunctionTemplateParamNamesFunctionTemplateParamKindsFunctionTemplateParamTypesFunctionTemplateParamValuesFunctionTemplateParamEnablesClassDeclClassTemplateSpecKindClassTemplateParamNamesClassTemplateParamKindsClassTemplateParamTypesClassTemplateParamValuesClassTemplateParamEnablesClassCtorDeclsClassCtorParamNamesClassCtorParamTypesClassCtorParamSerializedTypes[1 1]@C[28 1]@t6@filtert42@../../../aie/aie_kernels/FirDoubleStream.hC[4 1]@t4@sin1t4@sin2t3@cint4@coutC[4 1]@t30@input_stream_cint16 * restrictt30@input_stream_cint16 * restrictt26@input_stream< cacc48_t > *t27@output_stream< cacc48_t > *C[4 1]@t37@{Q2{P{Tinput_stream{1{t{Scint16}}}}}}t37@{Q2{P{Tinput_stream{1{t{Scint16}}}}}}t35@{P{Tinput_stream{1{t{Scacc48_t}}}}}t36@{P{Toutput_stream{1{t{Scacc48_t}}}}}C[4 1]@t5@inputt5@inputt5@inputt6@outputC[4 1]@l0@l0@l0@l0@C[4 1]@l0@l0@l0@l0@C[4 1]@l0@l0@l0@l0@C[4 1]@l0@l0@l0@l1@t281@namespace DoubleStream {
      | template < int NSamples, int ShiftAcc, bool DiscardSample, bool SwapRead > 
      | void FIR_MultiKernel_cincout::
      | filter(input_stream_cint16 * restrict sin1, input_stream_cint16 * restrict sin2, input_stream< cacc48_t > * cin, output_stream< cacc48_t > * cout);
      | }t4@nonee[0 1]@e[0 1]@e[0 1]@e[0 1]@e[0 1]@t132@namespace DoubleStream {
      | template < int NSamples, int ShiftAcc, bool DiscardSample, bool SwapRead > class FIR_MultiKernel_cincout;
      | }t8@implicitC[4 1]@t8@NSamplest8@ShiftAcct13@DiscardSamplet8@SwapReadC[4 1]@t7@nontypet7@nontypet7@nontypet7@nontypeC[4 1]@t3@intt3@intt4@boolt4@boolC[4 1]@nnnnC[4 1]@l1@l1@l1@l1@C[1 1]@t54@FIR_MultiKernel_cincout(cint16 const ( & taps ) [ 4 ])C[1 1]@C[1 1]@t4@tapsC[1 1]@C[1 1]@t23@cint16 const ( &) [ 4 ]C[1 1]@C[1 1]@t20@{R{Q1{C{Scint16}4}}}
      FunctionDecl=|
      | namespace DoubleStream {
      | template < int NSamples, int ShiftAcc, bool DiscardSample, bool SwapRead > 
      | void FIR_MultiKernel_cincout::
      | filter(input_stream_cint16 * restrict sin1, input_stream_cint16 * restrict sin2, input_stream< cacc48_t > * cin, output_stream< cacc48_t > * cout);
      | }
      ClassDeclTypeOptions=|
      | C[1 1]@t132@namespace DoubleStream {
      | template < int NSamples, int ShiftAcc, bool DiscardSample, bool SwapRead > class FIR_MultiKernel_cincout;
      | }
      ClassDecl=|
      | namespace DoubleStream {
      | template < int NSamples, int ShiftAcc, bool DiscardSample, bool SwapRead > class FIR_MultiKernel_cincout;
      | }
  filter6 : aieBasic/AIE Class Kernel  KernelAllAttrs=|  PortNames={'sin1'; 'sin2'; 'cin'; 'cout'}  PortSerializedTypes={'{Q2{P{Tinput_stream{1{t{Scint16}}}}}}'; '{Q2{P{Tinput_stream{1{t{Scint16}}}}}}'; '{P{Tinput_stream{1{t{Scacc48_t}}}}}'; '{P{Toutput_stream{1{t{Scacc48_t}}}}}'}  PortWindowSizes={0.000000000000000000e+00; 0.000000000000000000e+00; 0.000000000000000000e+00; 0.000000000000000000e+00}  PortWindowMargins={0.000000000000000000e+00; 0.000000000000000000e+00; 0.000000000000000000e+00; 0.000000000000000000e+00}  PortSynchronicities={'auto'; 'auto'; 'auto'; 'auto'}  PortSignalSizes={0.000000000000000000e+00; 0.000000000000000000e+00; 0.000000000000000000e+00; 8.000000000000000000e+00}  ClassTemplateSpecKind=implicit  ClassTemplateParamNames={'NSamples'; 'ShiftAcc'; 'DiscardSample'; 'SwapRead'}  ClassTemplateParamKinds={'nontype'; 'nontype'; 'nontype'; 'nontype'}  ClassTemplateParamTypes={'int'; 'int'; 'bool'; 'bool'}  ClassTemplateParamValues={'512', '15', '0', '0'}  ClassCtorParamNames={'taps'}  ClassCtorParamSerializedTypes={'{R{Q1{C{Scint16}4}}}'}  ClassCtorParamValues={'[146-91i 4086+5221i 237-54i -83-21i]'}  ClassIndex=1  ClassCtorIndex=1  ClassTabVisible=on  ClassTemplateParamsVisible=on  ClassCtorDeclVisible=on  ClassCtorParamsVisible=on  FunctionTabVisible=on  FunctionDecl=|  PortAttrs={ 'input', 'sin1', 'input_stream_cint16 * restrict', '', '', '', ''; 'input', 'sin2', 'input_stream_cint16 * restrict', '', '', '', ''; 'input', 'cin', 'input_stream< cacc48_t > *', '', '', '', ''; 'output', 'cout', 'output_stream< cacc48_t > *', '', '', '', 'OUTPUT_SIZE' }  PortAttrsEnables={'off', 'off', 'off', 'off', 'off', 'off', 'off';'off', 'off', 'off', 'off', 'off', 'off', 'off';'off', 'off', 'off', 'off', 'off', 'off', 'off';'off', 'off', 'off', 'off', 'off', 'off', 'on'}  SampleTime=-1  ClassDeclTypeOptions=|  ClassDecl=|  ClassTemplateParams={ 'NSamples', 'int', 'BURST_LENGTH'; 'ShiftAcc', 'int', 'SHIFT_ACC'; 'DiscardSample', 'bool', 'FALSE'; 'SwapRead', 'bool', 'FALSE' }  ClassTemplateParamsEnables={'off', 'off', 'on';'off', 'off', 'on';'off', 'off', 'on';'off', 'off', 'on'}  ClassCtorDeclTypeOptions=C[1 1]@t54@FIR_MultiKernel_cincout(cint16 const ( & taps ) [ 4 ])  ClassCtorDecl=FIR_MultiKernel_cincout(cint16 const ( & taps ) [ 4 ])  ClassCtorParams={ 'taps', 'cint16 const ( &) [ 4 ]', 'phi_6' }  KernelHeaderFile=FirDoubleStream.h  KernelClassName=DoubleStream::FIR_MultiKernel_cincout  KernelFunction=filter  KernelSourceFile=FirDoubleStream.cpp  KernelSearchPaths={'$SRC/aie_kernels'}  PreProcOptions={}  CoreRuntimeRatio=0.9  KernelLocSpec=off  ColRowLocation=[0 0]  blockJsonConstraints="{\"type\":\"constraint\",\"constraintType\":\"coreUtilization\",\"sid\":\"845\",\"lhs\":{\"type\":\"runtimeRatio\",\"args\":{\"type\":\"kernel\",\"name\":\"DualStreamSSR_b/Subsystem/filter6\",\"sid\":\"845\"}},\"rhs\":{\"type\":\"evaluable\",\"expr\":\"0.9\",\"value\":0.9},\"equality\":true}"  deprecateConstraints=1
      KernelAllAttrs=|
      | s[12;12;9;9;19;14;21;23;24;21;12;24;26;26;26;27;28;9;21;23;23;23;24;25;14;19;19;29]@FunctionNameDeclFileNamePortNamesPortTypesPortSerializedTypesPortDirectionsPortWindowSizeEnablesPortWindowMarginEnablesPortSynchronicityEnablesPortSignalSizeEnablesFunctionDeclFunctionTemplateSpecKindFunctionTemplateParamNamesFunctionTemplateParamKindsFunctionTemplateParamTypesFunctionTemplateParamValuesFunctionTemplateParamEnablesClassDeclClassTemplateSpecKindClassTemplateParamNamesClassTemplateParamKindsClassTemplateParamTypesClassTemplateParamValuesClassTemplateParamEnablesClassCtorDeclsClassCtorParamNamesClassCtorParamTypesClassCtorParamSerializedTypes[1 1]@C[28 1]@t6@filtert42@../../../aie/aie_kernels/FirDoubleStream.hC[4 1]@t4@sin1t4@sin2t3@cint4@coutC[4 1]@t30@input_stream_cint16 * restrictt30@input_stream_cint16 * restrictt26@input_stream< cacc48_t > *t27@output_stream< cacc48_t > *C[4 1]@t37@{Q2{P{Tinput_stream{1{t{Scint16}}}}}}t37@{Q2{P{Tinput_stream{1{t{Scint16}}}}}}t35@{P{Tinput_stream{1{t{Scacc48_t}}}}}t36@{P{Toutput_stream{1{t{Scacc48_t}}}}}C[4 1]@t5@inputt5@inputt5@inputt6@outputC[4 1]@l0@l0@l0@l0@C[4 1]@l0@l0@l0@l0@C[4 1]@l0@l0@l0@l0@C[4 1]@l0@l0@l0@l1@t281@namespace DoubleStream {
      | template < int NSamples, int ShiftAcc, bool DiscardSample, bool SwapRead > 
      | void FIR_MultiKernel_cincout::
      | filter(input_stream_cint16 * restrict sin1, input_stream_cint16 * restrict sin2, input_stream< cacc48_t > * cin, output_stream< cacc48_t > * cout);
      | }t4@nonee[0 1]@e[0 1]@e[0 1]@e[0 1]@e[0 1]@t132@namespace DoubleStream {
      | template < int NSamples, int ShiftAcc, bool DiscardSample, bool SwapRead > class FIR_MultiKernel_cincout;
      | }t8@implicitC[4 1]@t8@NSamplest8@ShiftAcct13@DiscardSamplet8@SwapReadC[4 1]@t7@nontypet7@nontypet7@nontypet7@nontypeC[4 1]@t3@intt3@intt4@boolt4@boolC[4 1]@nnnnC[4 1]@l1@l1@l1@l1@C[1 1]@t54@FIR_MultiKernel_cincout(cint16 const ( & taps ) [ 4 ])C[1 1]@C[1 1]@t4@tapsC[1 1]@C[1 1]@t23@cint16 const ( &) [ 4 ]C[1 1]@C[1 1]@t20@{R{Q1{C{Scint16}4}}}
      FunctionDecl=|
      | namespace DoubleStream {
      | template < int NSamples, int ShiftAcc, bool DiscardSample, bool SwapRead > 
      | void FIR_MultiKernel_cincout::
      | filter(input_stream_cint16 * restrict sin1, input_stream_cint16 * restrict sin2, input_stream< cacc48_t > * cin, output_stream< cacc48_t > * cout);
      | }
      ClassDeclTypeOptions=|
      | C[1 1]@t132@namespace DoubleStream {
      | template < int NSamples, int ShiftAcc, bool DiscardSample, bool SwapRead > class FIR_MultiKernel_cincout;
      | }
      ClassDecl=|
      | namespace DoubleStream {
      | template < int NSamples, int ShiftAcc, bool DiscardSample, bool SwapRead > class FIR_MultiKernel_cincout;
      | }
  filter60 : aieBasic/AIE Class Kernel  KernelAllAttrs=|  PortNames={'sin1'; 'sin2'; 'cin'; 'cout'}  PortSerializedTypes={'{Q2{P{Tinput_stream{1{t{Scint16}}}}}}'; '{Q2{P{Tinput_stream{1{t{Scint16}}}}}}'; '{P{Tinput_stream{1{t{Scacc48_t}}}}}'; '{P{Toutput_stream{1{t{Scacc48_t}}}}}'}  PortWindowSizes={0.000000000000000000e+00; 0.000000000000000000e+00; 0.000000000000000000e+00; 0.000000000000000000e+00}  PortWindowMargins={0.000000000000000000e+00; 0.000000000000000000e+00; 0.000000000000000000e+00; 0.000000000000000000e+00}  PortSynchronicities={'auto'; 'auto'; 'auto'; 'auto'}  PortSignalSizes={0.000000000000000000e+00; 0.000000000000000000e+00; 0.000000000000000000e+00; 8.000000000000000000e+00}  ClassTemplateSpecKind=implicit  ClassTemplateParamNames={'NSamples'; 'ShiftAcc'; 'DiscardSample'; 'SwapRead'}  ClassTemplateParamKinds={'nontype'; 'nontype'; 'nontype'; 'nontype'}  ClassTemplateParamTypes={'int'; 'int'; 'bool'; 'bool'}  ClassTemplateParamValues={'512', '15', '0', '0'}  ClassCtorParamNames={'taps'}  ClassCtorParamSerializedTypes={'{R{Q1{C{Scint16}4}}}'}  ClassCtorParamValues={'[-21+26i 1183+239i 248-2878i -160+111i]'}  ClassIndex=1  ClassCtorIndex=1  ClassTabVisible=on  ClassTemplateParamsVisible=on  ClassCtorDeclVisible=on  ClassCtorParamsVisible=on  FunctionTabVisible=on  FunctionDecl=|  PortAttrs={ 'input', 'sin1', 'input_stream_cint16 * restrict', '', '', '', ''; 'input', 'sin2', 'input_stream_cint16 * restrict', '', '', '', ''; 'input', 'cin', 'input_stream< cacc48_t > *', '', '', '', ''; 'output', 'cout', 'output_stream< cacc48_t > *', '', '', '', 'OUTPUT_SIZE' }  PortAttrsEnables={'off', 'off', 'off', 'off', 'off', 'off', 'off';'off', 'off', 'off', 'off', 'off', 'off', 'off';'off', 'off', 'off', 'off', 'off', 'off', 'off';'off', 'off', 'off', 'off', 'off', 'off', 'on'}  SampleTime=-1  ClassDeclTypeOptions=|  ClassDecl=|  ClassTemplateParams={ 'NSamples', 'int', 'BURST_LENGTH'; 'ShiftAcc', 'int', 'SHIFT_ACC'; 'DiscardSample', 'bool', 'FALSE'; 'SwapRead', 'bool', 'FALSE' }  ClassTemplateParamsEnables={'off', 'off', 'on';'off', 'off', 'on';'off', 'off', 'on';'off', 'off', 'on'}  ClassCtorDeclTypeOptions=C[1 1]@t54@FIR_MultiKernel_cincout(cint16 const ( & taps ) [ 4 ])  ClassCtorDecl=FIR_MultiKernel_cincout(cint16 const ( & taps ) [ 4 ])  ClassCtorParams={ 'taps', 'cint16 const ( &) [ 4 ]', 'phi_2' }  KernelHeaderFile=FirDoubleStream.h  KernelClassName=DoubleStream::FIR_MultiKernel_cincout  KernelFunction=filter  KernelSourceFile=FirDoubleStream.cpp  KernelSearchPaths={'$SRC/aie_kernels'}  PreProcOptions={}  CoreRuntimeRatio=0.9  KernelLocSpec=off  ColRowLocation=[0 0]  blockJsonConstraints="{\"type\":\"constraint\",\"constraintType\":\"coreUtilization\",\"sid\":\"846\",\"lhs\":{\"type\":\"runtimeRatio\",\"args\":{\"type\":\"kernel\",\"name\":\"DualStreamSSR_b/Subsystem/filter60\",\"sid\":\"846\"}},\"rhs\":{\"type\":\"evaluable\",\"expr\":\"0.9\",\"value\":0.9},\"equality\":true}"  deprecateConstraints=1
      KernelAllAttrs=|
      | s[12;12;9;9;19;14;21;23;24;21;12;24;26;26;26;27;28;9;21;23;23;23;24;25;14;19;19;29]@FunctionNameDeclFileNamePortNamesPortTypesPortSerializedTypesPortDirectionsPortWindowSizeEnablesPortWindowMarginEnablesPortSynchronicityEnablesPortSignalSizeEnablesFunctionDeclFunctionTemplateSpecKindFunctionTemplateParamNamesFunctionTemplateParamKindsFunctionTemplateParamTypesFunctionTemplateParamValuesFunctionTemplateParamEnablesClassDeclClassTemplateSpecKindClassTemplateParamNamesClassTemplateParamKindsClassTemplateParamTypesClassTemplateParamValuesClassTemplateParamEnablesClassCtorDeclsClassCtorParamNamesClassCtorParamTypesClassCtorParamSerializedTypes[1 1]@C[28 1]@t6@filtert42@../../../aie/aie_kernels/FirDoubleStream.hC[4 1]@t4@sin1t4@sin2t3@cint4@coutC[4 1]@t30@input_stream_cint16 * restrictt30@input_stream_cint16 * restrictt26@input_stream< cacc48_t > *t27@output_stream< cacc48_t > *C[4 1]@t37@{Q2{P{Tinput_stream{1{t{Scint16}}}}}}t37@{Q2{P{Tinput_stream{1{t{Scint16}}}}}}t35@{P{Tinput_stream{1{t{Scacc48_t}}}}}t36@{P{Toutput_stream{1{t{Scacc48_t}}}}}C[4 1]@t5@inputt5@inputt5@inputt6@outputC[4 1]@l0@l0@l0@l0@C[4 1]@l0@l0@l0@l0@C[4 1]@l0@l0@l0@l0@C[4 1]@l0@l0@l0@l1@t281@namespace DoubleStream {
      | template < int NSamples, int ShiftAcc, bool DiscardSample, bool SwapRead > 
      | void FIR_MultiKernel_cincout::
      | filter(input_stream_cint16 * restrict sin1, input_stream_cint16 * restrict sin2, input_stream< cacc48_t > * cin, output_stream< cacc48_t > * cout);
      | }t4@nonee[0 1]@e[0 1]@e[0 1]@e[0 1]@e[0 1]@t132@namespace DoubleStream {
      | template < int NSamples, int ShiftAcc, bool DiscardSample, bool SwapRead > class FIR_MultiKernel_cincout;
      | }t8@implicitC[4 1]@t8@NSamplest8@ShiftAcct13@DiscardSamplet8@SwapReadC[4 1]@t7@nontypet7@nontypet7@nontypet7@nontypeC[4 1]@t3@intt3@intt4@boolt4@boolC[4 1]@nnnnC[4 1]@l1@l1@l1@l1@C[1 1]@t54@FIR_MultiKernel_cincout(cint16 const ( & taps ) [ 4 ])C[1 1]@C[1 1]@t4@tapsC[1 1]@C[1 1]@t23@cint16 const ( &) [ 4 ]C[1 1]@C[1 1]@t20@{R{Q1{C{Scint16}4}}}
      FunctionDecl=|
      | namespace DoubleStream {
      | template < int NSamples, int ShiftAcc, bool DiscardSample, bool SwapRead > 
      | void FIR_MultiKernel_cincout::
      | filter(input_stream_cint16 * restrict sin1, input_stream_cint16 * restrict sin2, input_stream< cacc48_t > * cin, output_stream< cacc48_t > * cout);
      | }
      ClassDeclTypeOptions=|
      | C[1 1]@t132@namespace DoubleStream {
      | template < int NSamples, int ShiftAcc, bool DiscardSample, bool SwapRead > class FIR_MultiKernel_cincout;
      | }
      ClassDecl=|
      | namespace DoubleStream {
      | template < int NSamples, int ShiftAcc, bool DiscardSample, bool SwapRead > class FIR_MultiKernel_cincout;
      | }
  filter61 : aieBasic/AIE Class Kernel  KernelAllAttrs=|  PortNames={'sin1'; 'sin2'; 'cin'; 'sout1'; 'sout2'}  PortSerializedTypes={'{Q2{P{Tinput_stream{1{t{Scint16}}}}}}'; '{Q2{P{Tinput_stream{1{t{Scint16}}}}}}'; '{P{Tinput_stream{1{t{Scacc48_t}}}}}'; '{Q2{P{Toutput_stream{1{t{Scint16}}}}}}'; '{Q2{P{Toutput_stream{1{t{Scint16}}}}}}'}  PortWindowSizes={0.000000000000000000e+00; 0.000000000000000000e+00; 0.000000000000000000e+00; 0.000000000000000000e+00; 0.000000000000000000e+00}  PortWindowMargins={0.000000000000000000e+00; 0.000000000000000000e+00; 0.000000000000000000e+00; 0.000000000000000000e+00; 0.000000000000000000e+00}  PortSynchronicities={'auto'; 'auto'; 'auto'; 'auto'; 'auto'}  PortSignalSizes={0.000000000000000000e+00; 0.000000000000000000e+00; 0.000000000000000000e+00; 4.000000000000000000e+00; 4.000000000000000000e+00}  ClassTemplateSpecKind=implicit  ClassTemplateParamNames={'NSamples'; 'ShiftAcc'; 'DiscardSample'; 'SwapRead'}  ClassTemplateParamKinds={'nontype'; 'nontype'; 'nontype'; 'nontype'}  ClassTemplateParamTypes={'int'; 'int'; 'bool'; 'bool'}  ClassTemplateParamValues={'512', '15', '0', '0'}  ClassCtorParamNames={'taps'}  ClassCtorParamSerializedTypes={'{R{Q1{C{Scint16}4}}}'}  ClassCtorParamValues={'[14-121i 1454-497i 237+96i -121+233i]'}  ClassIndex=1  ClassCtorIndex=1  ClassTabVisible=on  ClassTemplateParamsVisible=on  ClassCtorDeclVisible=on  ClassCtorParamsVisible=on  FunctionTabVisible=on  FunctionDecl=|  PortAttrs={ 'input', 'sin1', 'input_stream_cint16 * restrict', '', '', '', ''; 'input', 'sin2', 'input_stream_cint16 * restrict', '', '', '', ''; 'input', 'cin', 'input_stream< cacc48_t > *', '', '', '', ''; 'output', 'sout1', 'output_stream_cint16 * restrict', '', '', '', 'OUTPUT_SIZE/2'; 'output', 'sout2', 'output_stream_cint16 * restrict', '', '', '', 'OUTPUT_SIZE/2' }  PortAttrsEnables={'off', 'off', 'off', 'off', 'off', 'off', 'off';'off', 'off', 'off', 'off', 'off', 'off', 'off';'off', 'off', 'off', 'off', 'off', 'off', 'off';'off', 'off', 'off', 'off', 'off', 'off', 'on';'off', 'off', 'off', 'off', 'off', 'off', 'on'}  SampleTime=-1  ClassDeclTypeOptions=|  ClassDecl=|  ClassTemplateParams={ 'NSamples', 'int', 'BURST_LENGTH'; 'ShiftAcc', 'int', 'SHIFT_ACC'; 'DiscardSample', 'bool', 'FALSE'; 'SwapRead', 'bool', 'FALSE' }  ClassTemplateParamsEnables={'off', 'off', 'on';'off', 'off', 'on';'off', 'off', 'on';'off', 'off', 'on'}  ClassCtorDeclTypeOptions=C[1 1]@t50@FIR_MultiKernel_cin(cint16 const ( & taps ) [ 4 ])  ClassCtorDecl=FIR_MultiKernel_cin(cint16 const ( & taps ) [ 4 ])  ClassCtorParams={ 'taps', 'cint16 const ( &) [ 4 ]', 'phi_3' }  KernelHeaderFile=FirDoubleStream.h  KernelClassName=DoubleStream::FIR_MultiKernel_cin  KernelFunction=filter  KernelSourceFile=FirDoubleStream.cpp  KernelSearchPaths={'$SRC/aie_kernels'}  PreProcOptions={}  CoreRuntimeRatio=0.9  KernelLocSpec=off  ColRowLocation=[0 0]  blockJsonConstraints="{\"type\":\"constraint\",\"constraintType\":\"coreUtilization\",\"sid\":\"847\",\"lhs\":{\"type\":\"runtimeRatio\",\"args\":{\"type\":\"kernel\",\"name\":\"DualStreamSSR_b/Subsystem/filter61\",\"sid\":\"847\"}},\"rhs\":{\"type\":\"evaluable\",\"expr\":\"0.9\",\"value\":0.9},\"equality\":true}"  deprecateConstraints=1
      KernelAllAttrs=|
      | s[12;12;9;9;19;14;21;23;24;21;12;24;26;26;26;27;28;9;21;23;23;23;24;25;14;19;19;29]@FunctionNameDeclFileNamePortNamesPortTypesPortSerializedTypesPortDirectionsPortWindowSizeEnablesPortWindowMarginEnablesPortSynchronicityEnablesPortSignalSizeEnablesFunctionDeclFunctionTemplateSpecKindFunctionTemplateParamNamesFunctionTemplateParamKindsFunctionTemplateParamTypesFunctionTemplateParamValuesFunctionTemplateParamEnablesClassDeclClassTemplateSpecKindClassTemplateParamNamesClassTemplateParamKindsClassTemplateParamTypesClassTemplateParamValuesClassTemplateParamEnablesClassCtorDeclsClassCtorParamNamesClassCtorParamTypesClassCtorParamSerializedTypes[1 1]@C[28 1]@t6@filtert42@../../../aie/aie_kernels/FirDoubleStream.hC[5 1]@t4@sin1t4@sin2t3@cint5@sout1t5@sout2C[5 1]@t30@input_stream_cint16 * restrictt30@input_stream_cint16 * restrictt26@input_stream< cacc48_t > *t31@output_stream_cint16 * restrictt31@output_stream_cint16 * restrictC[5 1]@t37@{Q2{P{Tinput_stream{1{t{Scint16}}}}}}t37@{Q2{P{Tinput_stream{1{t{Scint16}}}}}}t35@{P{Tinput_stream{1{t{Scacc48_t}}}}}t38@{Q2{P{Toutput_stream{1{t{Scint16}}}}}}t38@{Q2{P{Toutput_stream{1{t{Scint16}}}}}}C[5 1]@t5@inputt5@inputt5@inputt6@outputt6@outputC[5 1]@l0@l0@l0@l0@l0@C[5 1]@l0@l0@l0@l0@l0@C[5 1]@l0@l0@l0@l0@l0@C[5 1]@l0@l0@l0@l1@l1@t321@namespace DoubleStream {
      | template < int NSamples, int ShiftAcc, bool DiscardSample, bool SwapRead > 
      | void FIR_MultiKernel_cin::
      | filter(input_stream_cint16 * restrict sin1, input_stream_cint16 * restrict sin2, input_stream< cacc48_t > * cin, output_stream_cint16 * restrict sout1, output_stream_cint16 * restrict sout2);
      | }t4@nonee[0 1]@e[0 1]@e[0 1]@e[0 1]@e[0 1]@t128@namespace DoubleStream {
      | template < int NSamples, int ShiftAcc, bool DiscardSample, bool SwapRead > class FIR_MultiKernel_cin;
      | }t8@implicitC[4 1]@t8@NSamplest8@ShiftAcct13@DiscardSamplet8@SwapReadC[4 1]@t7@nontypet7@nontypet7@nontypet7@nontypeC[4 1]@t3@intt3@intt4@boolt4@boolC[4 1]@nnnnC[4 1]@l1@l1@l1@l1@C[1 1]@t50@FIR_MultiKernel_cin(cint16 const ( & taps ) [ 4 ])C[1 1]@C[1 1]@t4@tapsC[1 1]@C[1 1]@t23@cint16 const ( &) [ 4 ]C[1 1]@C[1 1]@t20@{R{Q1{C{Scint16}4}}}
      FunctionDecl=|
      | namespace DoubleStream {
      | template < int NSamples, int ShiftAcc, bool DiscardSample, bool SwapRead > 
      | void FIR_MultiKernel_cin::
      | filter(input_stream_cint16 * restrict sin1, input_stream_cint16 * restrict sin2, input_stream< cacc48_t > * cin, output_stream_cint16 * restrict sout1, output_stream_cint16 * restrict sout2);
      | }
      ClassDeclTypeOptions=|
      | C[1 1]@t128@namespace DoubleStream {
      | template < int NSamples, int ShiftAcc, bool DiscardSample, bool SwapRead > class FIR_MultiKernel_cin;
      | }
      ClassDecl=|
      | namespace DoubleStream {
      | template < int NSamples, int ShiftAcc, bool DiscardSample, bool SwapRead > class FIR_MultiKernel_cin;
      | }
  filter62 : aieBasic/AIE Class Kernel  KernelAllAttrs=|  PortNames={'sin1'; 'sin2'; 'cout'}  PortSerializedTypes={'{Q2{P{Tinput_stream{1{t{Scint16}}}}}}'; '{Q2{P{Tinput_stream{1{t{Scint16}}}}}}'; '{P{Toutput_stream{1{t{Scacc48_t}}}}}'}  PortWindowSizes={0.000000000000000000e+00; 0.000000000000000000e+00; 0.000000000000000000e+00}  PortWindowMargins={0.000000000000000000e+00; 0.000000000000000000e+00; 0.000000000000000000e+00}  PortSynchronicities={'auto'; 'auto'; 'auto'}  PortSignalSizes={0.000000000000000000e+00; 0.000000000000000000e+00; 8.000000000000000000e+00}  ClassTemplateSpecKind=implicit  ClassTemplateParamNames={'NSamples'; 'ShiftAcc'; 'DiscardSample'; 'SwapRead'}  ClassTemplateParamKinds={'nontype'; 'nontype'; 'nontype'; 'nontype'}  ClassTemplateParamTypes={'int'; 'int'; 'bool'; 'bool'}  ClassTemplateParamValues={'512', '15', '0', '0'}  ClassCtorParamNames={'taps'}  ClassCtorParamSerializedTypes={'{R{Q1{C{Scint16}4}}}'}  ClassCtorParamValues={'[-21+26i 1183+239i 248-2878i -160+111i]'}  ClassIndex=1  ClassCtorIndex=1  ClassTabVisible=on  ClassTemplateParamsVisible=on  ClassCtorDeclVisible=on  ClassCtorParamsVisible=on  FunctionTabVisible=on  FunctionDecl=|  PortAttrs={ 'input', 'sin1', 'input_stream_cint16 * restrict', '', '', '', ''; 'input', 'sin2', 'input_stream_cint16 * restrict', '', '', '', ''; 'output', 'cout', 'output_stream< cacc48_t > *', '', '', '', 'OUTPUT_SIZE' }  PortAttrsEnables={'off', 'off', 'off', 'off', 'off', 'off', 'off';'off', 'off', 'off', 'off', 'off', 'off', 'off';'off', 'off', 'off', 'off', 'off', 'off', 'on'}  SampleTime=-1  ClassDeclTypeOptions=|  ClassDecl=|  ClassTemplateParams={ 'NSamples', 'int', 'BURST_LENGTH'; 'ShiftAcc', 'int', 'SHIFT_ACC'; 'DiscardSample', 'bool', 'FALSE'; 'SwapRead', 'bool', 'FALSE' }  ClassTemplateParamsEnables={'off', 'off', 'on';'off', 'off', 'on';'off', 'off', 'on';'off', 'off', 'on'}  ClassCtorDeclTypeOptions=C[1 1]@t51@FIR_MultiKernel_cout(cint16 const ( & taps ) [ 4 ])  ClassCtorDecl=FIR_MultiKernel_cout(cint16 const ( & taps ) [ 4 ])  ClassCtorParams={ 'taps', 'cint16 const ( &) [ 4 ]', 'phi_2' }  KernelHeaderFile=FirDoubleStream.h  KernelClassName=DoubleStream::FIR_MultiKernel_cout  KernelFunction=filter  KernelSourceFile=FirDoubleStream.cpp  KernelSearchPaths={'$SRC/aie_kernels'}  PreProcOptions={}  CoreRuntimeRatio=0.9  KernelLocSpec=off  ColRowLocation=[0 0]  blockJsonConstraints="[{\"type\":\"constraint\",\"constraintType\":\"coreUtilization\",\"sid\":\"848\",\"lhs\":{\"type\":\"runtimeRatio\",\"args\":{\"type\":\"kernel\",\"name\":\"DualStreamSSR/SSR8/filter62\",\"sid\":\"848\"}},\"rhs\":{\"type\":\"evaluable\",\"expr\":\"0.9\",\"value\":0.9},\"equality\":true},{\"type\":\"constraint\",\"constraintType\":\"location_kernel\",\"sid\":\"848\",\"lhs\":{\"type\":\"location\",\"templParam\":\"kernel\",\"args\":{\"type\":\"kernel\",\"name\":\"DualStreamSSR/SSR8/filter62\",\"sid\":\"848\"}},\"rhs\":{\"type\":\"tile\",\"args\":[{\"type\":\"evaluable\",\"expr\":\"30\",\"value\":30},{\"type\":\"evaluable\",\"expr\":\"5\",\"value\":5}]},\"equality\":true}]"  deprecateConstraints=1
      KernelAllAttrs=|
      | s[12;12;9;9;19;14;21;23;24;21;12;24;26;26;26;27;28;9;21;23;23;23;24;25;14;19;19;29]@FunctionNameDeclFileNamePortNamesPortTypesPortSerializedTypesPortDirectionsPortWindowSizeEnablesPortWindowMarginEnablesPortSynchronicityEnablesPortSignalSizeEnablesFunctionDeclFunctionTemplateSpecKindFunctionTemplateParamNamesFunctionTemplateParamKindsFunctionTemplateParamTypesFunctionTemplateParamValuesFunctionTemplateParamEnablesClassDeclClassTemplateSpecKindClassTemplateParamNamesClassTemplateParamKindsClassTemplateParamTypesClassTemplateParamValuesClassTemplateParamEnablesClassCtorDeclsClassCtorParamNamesClassCtorParamTypesClassCtorParamSerializedTypes[1 1]@C[28 1]@t6@filtert42@../../../aie/aie_kernels/FirDoubleStream.hC[3 1]@t4@sin1t4@sin2t4@coutC[3 1]@t30@input_stream_cint16 * restrictt30@input_stream_cint16 * restrictt27@output_stream< cacc48_t > *C[3 1]@t37@{Q2{P{Tinput_stream{1{t{Scint16}}}}}}t37@{Q2{P{Tinput_stream{1{t{Scint16}}}}}}t36@{P{Toutput_stream{1{t{Scacc48_t}}}}}C[3 1]@t5@inputt5@inputt6@outputC[3 1]@l0@l0@l0@C[3 1]@l0@l0@l0@C[3 1]@l0@l0@l0@C[3 1]@l0@l0@l1@t246@namespace DoubleStream {
      | template < int NSamples, int ShiftAcc, bool DiscardSample, bool SwapRead > 
      | void FIR_MultiKernel_cout::
      | filter(input_stream_cint16 * restrict sin1, input_stream_cint16 * restrict sin2, output_stream< cacc48_t > * cout);
      | }t4@nonee[0 1]@e[0 1]@e[0 1]@e[0 1]@e[0 1]@t129@namespace DoubleStream {
      | template < int NSamples, int ShiftAcc, bool DiscardSample, bool SwapRead > class FIR_MultiKernel_cout;
      | }t8@implicitC[4 1]@t8@NSamplest8@ShiftAcct13@DiscardSamplet8@SwapReadC[4 1]@t7@nontypet7@nontypet7@nontypet7@nontypeC[4 1]@t3@intt3@intt4@boolt4@boolC[4 1]@nnnnC[4 1]@l1@l1@l1@l1@C[1 1]@t51@FIR_MultiKernel_cout(cint16 const ( & taps ) [ 4 ])C[1 1]@C[1 1]@t4@tapsC[1 1]@C[1 1]@t23@cint16 const ( &) [ 4 ]C[1 1]@C[1 1]@t20@{R{Q1{C{Scint16}4}}}
      FunctionDecl=|
      | namespace DoubleStream {
      | template < int NSamples, int ShiftAcc, bool DiscardSample, bool SwapRead > 
      | void FIR_MultiKernel_cout::
      | filter(input_stream_cint16 * restrict sin1, input_stream_cint16 * restrict sin2, output_stream< cacc48_t > * cout);
      | }
      ClassDeclTypeOptions=|
      | C[1 1]@t129@namespace DoubleStream {
      | template < int NSamples, int ShiftAcc, bool DiscardSample, bool SwapRead > class FIR_MultiKernel_cout;
      | }
      ClassDecl=|
      | namespace DoubleStream {
      | template < int NSamples, int ShiftAcc, bool DiscardSample, bool SwapRead > class FIR_MultiKernel_cout;
      | }
  filter63 : aieBasic/AIE Class Kernel  KernelAllAttrs=|  PortNames={'sin1'; 'sin2'; 'cin'; 'cout'}  PortSerializedTypes={'{Q2{P{Tinput_stream{1{t{Scint16}}}}}}'; '{Q2{P{Tinput_stream{1{t{Scint16}}}}}}'; '{P{Tinput_stream{1{t{Scacc48_t}}}}}'; '{P{Toutput_stream{1{t{Scacc48_t}}}}}'}  PortWindowSizes={0.000000000000000000e+00; 0.000000000000000000e+00; 0.000000000000000000e+00; 0.000000000000000000e+00}  PortWindowMargins={0.000000000000000000e+00; 0.000000000000000000e+00; 0.000000000000000000e+00; 0.000000000000000000e+00}  PortSynchronicities={'auto'; 'auto'; 'auto'; 'auto'}  PortSignalSizes={0.000000000000000000e+00; 0.000000000000000000e+00; 0.000000000000000000e+00; 8.000000000000000000e+00}  ClassTemplateSpecKind=implicit  ClassTemplateParamNames={'NSamples'; 'ShiftAcc'; 'DiscardSample'; 'SwapRead'}  ClassTemplateParamKinds={'nontype'; 'nontype'; 'nontype'; 'nontype'}  ClassTemplateParamTypes={'int'; 'int'; 'bool'; 'bool'}  ClassTemplateParamValues={'512', '15', '0', '0'}  ClassCtorParamNames={'taps'}  ClassCtorParamSerializedTypes={'{R{Q1{C{Scint16}4}}}'}  ClassCtorParamValues={'[-83+21i 237+54i 4086-5221i 146+91i]'}  ClassIndex=1  ClassCtorIndex=1  ClassTabVisible=on  ClassTemplateParamsVisible=on  ClassCtorDeclVisible=on  ClassCtorParamsVisible=on  FunctionTabVisible=on  FunctionDecl=|  PortAttrs={ 'input', 'sin1', 'input_stream_cint16 * restrict', '', '', '', ''; 'input', 'sin2', 'input_stream_cint16 * restrict', '', '', '', ''; 'input', 'cin', 'input_stream< cacc48_t > *', '', '', '', ''; 'output', 'cout', 'output_stream< cacc48_t > *', '', '', '', 'OUTPUT_SIZE' }  PortAttrsEnables={'off', 'off', 'off', 'off', 'off', 'off', 'off';'off', 'off', 'off', 'off', 'off', 'off', 'off';'off', 'off', 'off', 'off', 'off', 'off', 'off';'off', 'off', 'off', 'off', 'off', 'off', 'on'}  SampleTime=-1  ClassDeclTypeOptions=|  ClassDecl=|  ClassTemplateParams={ 'NSamples', 'int', 'BURST_LENGTH'; 'ShiftAcc', 'int', 'SHIFT_ACC'; 'DiscardSample', 'bool', 'FALSE'; 'SwapRead', 'bool', 'FALSE' }  ClassTemplateParamsEnables={'off', 'off', 'on';'off', 'off', 'on';'off', 'off', 'on';'off', 'off', 'on'}  ClassCtorDeclTypeOptions=C[1 1]@t54@FIR_MultiKernel_cincout(cint16 const ( & taps ) [ 4 ])  ClassCtorDecl=FIR_MultiKernel_cincout(cint16 const ( & taps ) [ 4 ])  ClassCtorParams={ 'taps', 'cint16 const ( &) [ 4 ]', 'phi_1' }  KernelHeaderFile=FirDoubleStream.h  KernelClassName=DoubleStream::FIR_MultiKernel_cincout  KernelFunction=filter  KernelSourceFile=FirDoubleStream.cpp  KernelSearchPaths={'$SRC/aie_kernels'}  PreProcOptions={}  CoreRuntimeRatio=0.9  KernelLocSpec=off  ColRowLocation=[0 0]  blockJsonConstraints="{\"type\":\"constraint\",\"constraintType\":\"coreUtilization\",\"sid\":\"849\",\"lhs\":{\"type\":\"runtimeRatio\",\"args\":{\"type\":\"kernel\",\"name\":\"DualStreamSSR_b/Subsystem/filter63\",\"sid\":\"849\"}},\"rhs\":{\"type\":\"evaluable\",\"expr\":\"0.9\",\"value\":0.9},\"equality\":true}"  deprecateConstraints=1
      KernelAllAttrs=|
      | s[12;12;9;9;19;14;21;23;24;21;12;24;26;26;26;27;28;9;21;23;23;23;24;25;14;19;19;29]@FunctionNameDeclFileNamePortNamesPortTypesPortSerializedTypesPortDirectionsPortWindowSizeEnablesPortWindowMarginEnablesPortSynchronicityEnablesPortSignalSizeEnablesFunctionDeclFunctionTemplateSpecKindFunctionTemplateParamNamesFunctionTemplateParamKindsFunctionTemplateParamTypesFunctionTemplateParamValuesFunctionTemplateParamEnablesClassDeclClassTemplateSpecKindClassTemplateParamNamesClassTemplateParamKindsClassTemplateParamTypesClassTemplateParamValuesClassTemplateParamEnablesClassCtorDeclsClassCtorParamNamesClassCtorParamTypesClassCtorParamSerializedTypes[1 1]@C[28 1]@t6@filtert42@../../../aie/aie_kernels/FirDoubleStream.hC[4 1]@t4@sin1t4@sin2t3@cint4@coutC[4 1]@t30@input_stream_cint16 * restrictt30@input_stream_cint16 * restrictt26@input_stream< cacc48_t > *t27@output_stream< cacc48_t > *C[4 1]@t37@{Q2{P{Tinput_stream{1{t{Scint16}}}}}}t37@{Q2{P{Tinput_stream{1{t{Scint16}}}}}}t35@{P{Tinput_stream{1{t{Scacc48_t}}}}}t36@{P{Toutput_stream{1{t{Scacc48_t}}}}}C[4 1]@t5@inputt5@inputt5@inputt6@outputC[4 1]@l0@l0@l0@l0@C[4 1]@l0@l0@l0@l0@C[4 1]@l0@l0@l0@l0@C[4 1]@l0@l0@l0@l1@t281@namespace DoubleStream {
      | template < int NSamples, int ShiftAcc, bool DiscardSample, bool SwapRead > 
      | void FIR_MultiKernel_cincout::
      | filter(input_stream_cint16 * restrict sin1, input_stream_cint16 * restrict sin2, input_stream< cacc48_t > * cin, output_stream< cacc48_t > * cout);
      | }t4@nonee[0 1]@e[0 1]@e[0 1]@e[0 1]@e[0 1]@t132@namespace DoubleStream {
      | template < int NSamples, int ShiftAcc, bool DiscardSample, bool SwapRead > class FIR_MultiKernel_cincout;
      | }t8@implicitC[4 1]@t8@NSamplest8@ShiftAcct13@DiscardSamplet8@SwapReadC[4 1]@t7@nontypet7@nontypet7@nontypet7@nontypeC[4 1]@t3@intt3@intt4@boolt4@boolC[4 1]@nnnnC[4 1]@l1@l1@l1@l1@C[1 1]@t54@FIR_MultiKernel_cincout(cint16 const ( & taps ) [ 4 ])C[1 1]@C[1 1]@t4@tapsC[1 1]@C[1 1]@t23@cint16 const ( &) [ 4 ]C[1 1]@C[1 1]@t20@{R{Q1{C{Scint16}4}}}
      FunctionDecl=|
      | namespace DoubleStream {
      | template < int NSamples, int ShiftAcc, bool DiscardSample, bool SwapRead > 
      | void FIR_MultiKernel_cincout::
      | filter(input_stream_cint16 * restrict sin1, input_stream_cint16 * restrict sin2, input_stream< cacc48_t > * cin, output_stream< cacc48_t > * cout);
      | }
      ClassDeclTypeOptions=|
      | C[1 1]@t132@namespace DoubleStream {
      | template < int NSamples, int ShiftAcc, bool DiscardSample, bool SwapRead > class FIR_MultiKernel_cincout;
      | }
      ClassDecl=|
      | namespace DoubleStream {
      | template < int NSamples, int ShiftAcc, bool DiscardSample, bool SwapRead > class FIR_MultiKernel_cincout;
      | }
  filter7 : aieBasic/AIE Class Kernel  KernelAllAttrs=|  PortNames={'sin1'; 'sin2'; 'cin'; 'sout1'; 'sout2'}  PortSerializedTypes={'{Q2{P{Tinput_stream{1{t{Scint16}}}}}}'; '{Q2{P{Tinput_stream{1{t{Scint16}}}}}}'; '{P{Tinput_stream{1{t{Scacc48_t}}}}}'; '{Q2{P{Toutput_stream{1{t{Scint16}}}}}}'; '{Q2{P{Toutput_stream{1{t{Scint16}}}}}}'}  PortWindowSizes={0.000000000000000000e+00; 0.000000000000000000e+00; 0.000000000000000000e+00; 0.000000000000000000e+00; 0.000000000000000000e+00}  PortWindowMargins={0.000000000000000000e+00; 0.000000000000000000e+00; 0.000000000000000000e+00; 0.000000000000000000e+00; 0.000000000000000000e+00}  PortSynchronicities={'auto'; 'auto'; 'auto'; 'auto'; 'auto'}  PortSignalSizes={0.000000000000000000e+00; 0.000000000000000000e+00; 0.000000000000000000e+00; 4.000000000000000000e+00; 4.000000000000000000e+00}  ClassTemplateSpecKind=implicit  ClassTemplateParamNames={'NSamples'; 'ShiftAcc'; 'DiscardSample'; 'SwapRead'}  ClassTemplateParamKinds={'nontype'; 'nontype'; 'nontype'; 'nontype'}  ClassTemplateParamTypes={'int'; 'int'; 'bool'; 'bool'}  ClassTemplateParamValues={'512', '15', '0', '0'}  ClassCtorParamNames={'taps'}  ClassCtorParamSerializedTypes={'{R{Q1{C{Scint16}4}}}'}  ClassCtorParamValues={'[342-439i 8773+2748i 102+525i -54+21i]'}  ClassIndex=1  ClassCtorIndex=1  ClassTabVisible=on  ClassTemplateParamsVisible=on  ClassCtorDeclVisible=on  ClassCtorParamsVisible=on  FunctionTabVisible=on  FunctionDecl=|  PortAttrs={ 'input', 'sin1', 'input_stream_cint16 * restrict', '', '', '', ''; 'input', 'sin2', 'input_stream_cint16 * restrict', '', '', '', ''; 'input', 'cin', 'input_stream< cacc48_t > *', '', '', '', ''; 'output', 'sout1', 'output_stream_cint16 * restrict', '', '', '', 'OUTPUT_SIZE/2'; 'output', 'sout2', 'output_stream_cint16 * restrict', '', '', '', 'OUTPUT_SIZE/2' }  PortAttrsEnables={'off', 'off', 'off', 'off', 'off', 'off', 'off';'off', 'off', 'off', 'off', 'off', 'off', 'off';'off', 'off', 'off', 'off', 'off', 'off', 'off';'off', 'off', 'off', 'off', 'off', 'off', 'on';'off', 'off', 'off', 'off', 'off', 'off', 'on'}  SampleTime=-1  ClassDeclTypeOptions=|  ClassDecl=|  ClassTemplateParams={ 'NSamples', 'int', 'BURST_LENGTH'; 'ShiftAcc', 'int', 'SHIFT_ACC'; 'DiscardSample', 'bool', 'FALSE'; 'SwapRead', 'bool', 'FALSE' }  ClassTemplateParamsEnables={'off', 'off', 'on';'off', 'off', 'on';'off', 'off', 'on';'off', 'off', 'on'}  ClassCtorDeclTypeOptions=C[1 1]@t50@FIR_MultiKernel_cin(cint16 const ( & taps ) [ 4 ])  ClassCtorDecl=FIR_MultiKernel_cin(cint16 const ( & taps ) [ 4 ])  ClassCtorParams={ 'taps', 'cint16 const ( &) [ 4 ]', 'phi_7' }  KernelHeaderFile=FirDoubleStream.h  KernelClassName=DoubleStream::FIR_MultiKernel_cin  KernelFunction=filter  KernelSourceFile=FirDoubleStream.cpp  KernelSearchPaths={'$SRC/aie_kernels'}  PreProcOptions={}  CoreRuntimeRatio=0.9  KernelLocSpec=off  ColRowLocation=[0 0]  blockJsonConstraints="{\"type\":\"constraint\",\"constraintType\":\"coreUtilization\",\"sid\":\"850\",\"lhs\":{\"type\":\"runtimeRatio\",\"args\":{\"type\":\"kernel\",\"name\":\"DualStreamSSR_b/Subsystem/filter7\",\"sid\":\"850\"}},\"rhs\":{\"type\":\"evaluable\",\"expr\":\"0.9\",\"value\":0.9},\"equality\":true}"  deprecateConstraints=1
      KernelAllAttrs=|
      | s[12;12;9;9;19;14;21;23;24;21;12;24;26;26;26;27;28;9;21;23;23;23;24;25;14;19;19;29]@FunctionNameDeclFileNamePortNamesPortTypesPortSerializedTypesPortDirectionsPortWindowSizeEnablesPortWindowMarginEnablesPortSynchronicityEnablesPortSignalSizeEnablesFunctionDeclFunctionTemplateSpecKindFunctionTemplateParamNamesFunctionTemplateParamKindsFunctionTemplateParamTypesFunctionTemplateParamValuesFunctionTemplateParamEnablesClassDeclClassTemplateSpecKindClassTemplateParamNamesClassTemplateParamKindsClassTemplateParamTypesClassTemplateParamValuesClassTemplateParamEnablesClassCtorDeclsClassCtorParamNamesClassCtorParamTypesClassCtorParamSerializedTypes[1 1]@C[28 1]@t6@filtert42@../../../aie/aie_kernels/FirDoubleStream.hC[5 1]@t4@sin1t4@sin2t3@cint5@sout1t5@sout2C[5 1]@t30@input_stream_cint16 * restrictt30@input_stream_cint16 * restrictt26@input_stream< cacc48_t > *t31@output_stream_cint16 * restrictt31@output_stream_cint16 * restrictC[5 1]@t37@{Q2{P{Tinput_stream{1{t{Scint16}}}}}}t37@{Q2{P{Tinput_stream{1{t{Scint16}}}}}}t35@{P{Tinput_stream{1{t{Scacc48_t}}}}}t38@{Q2{P{Toutput_stream{1{t{Scint16}}}}}}t38@{Q2{P{Toutput_stream{1{t{Scint16}}}}}}C[5 1]@t5@inputt5@inputt5@inputt6@outputt6@outputC[5 1]@l0@l0@l0@l0@l0@C[5 1]@l0@l0@l0@l0@l0@C[5 1]@l0@l0@l0@l0@l0@C[5 1]@l0@l0@l0@l1@l1@t321@namespace DoubleStream {
      | template < int NSamples, int ShiftAcc, bool DiscardSample, bool SwapRead > 
      | void FIR_MultiKernel_cin::
      | filter(input_stream_cint16 * restrict sin1, input_stream_cint16 * restrict sin2, input_stream< cacc48_t > * cin, output_stream_cint16 * restrict sout1, output_stream_cint16 * restrict sout2);
      | }t4@nonee[0 1]@e[0 1]@e[0 1]@e[0 1]@e[0 1]@t128@namespace DoubleStream {
      | template < int NSamples, int ShiftAcc, bool DiscardSample, bool SwapRead > class FIR_MultiKernel_cin;
      | }t8@implicitC[4 1]@t8@NSamplest8@ShiftAcct13@DiscardSamplet8@SwapReadC[4 1]@t7@nontypet7@nontypet7@nontypet7@nontypeC[4 1]@t3@intt3@intt4@boolt4@boolC[4 1]@nnnnC[4 1]@l1@l1@l1@l1@C[1 1]@t50@FIR_MultiKernel_cin(cint16 const ( & taps ) [ 4 ])C[1 1]@C[1 1]@t4@tapsC[1 1]@C[1 1]@t23@cint16 const ( &) [ 4 ]C[1 1]@C[1 1]@t20@{R{Q1{C{Scint16}4}}}
      FunctionDecl=|
      | namespace DoubleStream {
      | template < int NSamples, int ShiftAcc, bool DiscardSample, bool SwapRead > 
      | void FIR_MultiKernel_cin::
      | filter(input_stream_cint16 * restrict sin1, input_stream_cint16 * restrict sin2, input_stream< cacc48_t > * cin, output_stream_cint16 * restrict sout1, output_stream_cint16 * restrict sout2);
      | }
      ClassDeclTypeOptions=|
      | C[1 1]@t128@namespace DoubleStream {
      | template < int NSamples, int ShiftAcc, bool DiscardSample, bool SwapRead > class FIR_MultiKernel_cin;
      | }
      ClassDecl=|
      | namespace DoubleStream {
      | template < int NSamples, int ShiftAcc, bool DiscardSample, bool SwapRead > class FIR_MultiKernel_cin;
      | }
  filter8 : aieBasic/AIE Class Kernel  KernelAllAttrs=|  PortNames={'sin1'; 'sin2'; 'cout'}  PortSerializedTypes={'{Q2{P{Tinput_stream{1{t{Scint16}}}}}}'; '{Q2{P{Tinput_stream{1{t{Scint16}}}}}}'; '{P{Toutput_stream{1{t{Scacc48_t}}}}}'}  PortWindowSizes={0.000000000000000000e+00; 0.000000000000000000e+00; 0.000000000000000000e+00}  PortWindowMargins={0.000000000000000000e+00; 0.000000000000000000e+00; 0.000000000000000000e+00}  PortSynchronicities={'auto'; 'auto'; 'auto'}  PortSignalSizes={0.000000000000000000e+00; 0.000000000000000000e+00; 8.000000000000000000e+00}  ClassTemplateSpecKind=implicit  ClassTemplateParamNames={'NSamples'; 'ShiftAcc'; 'DiscardSample'; 'SwapRead'}  ClassTemplateParamKinds={'nontype'; 'nontype'; 'nontype'; 'nontype'}  ClassTemplateParamTypes={'int'; 'int'; 'bool'; 'bool'}  ClassTemplateParamValues={'512', '15', '0', '0'}  ClassCtorParamNames={'taps'}  ClassCtorParamSerializedTypes={'{R{Q1{C{Scint16}4}}}'}  ClassCtorParamValues={'[146-91i 4086+5221i 237-54i -83-21i]'}  ClassIndex=1  ClassCtorIndex=1  ClassTabVisible=on  ClassTemplateParamsVisible=on  ClassCtorDeclVisible=on  ClassCtorParamsVisible=on  FunctionTabVisible=on  FunctionDecl=|  PortAttrs={ 'input', 'sin1', 'input_stream_cint16 * restrict', '', '', '', ''; 'input', 'sin2', 'input_stream_cint16 * restrict', '', '', '', ''; 'output', 'cout', 'output_stream< cacc48_t > *', '', '', '', 'OUTPUT_SIZE' }  PortAttrsEnables={'off', 'off', 'off', 'off', 'off', 'off', 'off';'off', 'off', 'off', 'off', 'off', 'off', 'off';'off', 'off', 'off', 'off', 'off', 'off', 'on'}  SampleTime=-1  ClassDeclTypeOptions=|  ClassDecl=|  ClassTemplateParams={ 'NSamples', 'int', 'BURST_LENGTH'; 'ShiftAcc', 'int', 'SHIFT_ACC'; 'DiscardSample', 'bool', 'FALSE'; 'SwapRead', 'bool', 'FALSE' }  ClassTemplateParamsEnables={'off', 'off', 'on';'off', 'off', 'on';'off', 'off', 'on';'off', 'off', 'on'}  ClassCtorDeclTypeOptions=C[1 1]@t51@FIR_MultiKernel_cout(cint16 const ( & taps ) [ 4 ])  ClassCtorDecl=FIR_MultiKernel_cout(cint16 const ( & taps ) [ 4 ])  ClassCtorParams={ 'taps', 'cint16 const ( &) [ 4 ]', 'phi_6' }  KernelHeaderFile=FirDoubleStream.h  KernelClassName=DoubleStream::FIR_MultiKernel_cout  KernelFunction=filter  KernelSourceFile=FirDoubleStream.cpp  KernelSearchPaths={'$SRC/aie_kernels'}  PreProcOptions={}  CoreRuntimeRatio=0.9  KernelLocSpec=off  ColRowLocation=[0 0]  blockJsonConstraints="[{\"type\":\"constraint\",\"constraintType\":\"coreUtilization\",\"sid\":\"851\",\"lhs\":{\"type\":\"runtimeRatio\",\"args\":{\"type\":\"kernel\",\"name\":\"DualStreamSSR/SSR8/filter8\",\"sid\":\"851\"}},\"rhs\":{\"type\":\"evaluable\",\"expr\":\"0.9\",\"value\":0.9},\"equality\":true},{\"type\":\"constraint\",\"constraintType\":\"location_kernel\",\"sid\":\"851\",\"lhs\":{\"type\":\"location\",\"templParam\":\"kernel\",\"args\":{\"type\":\"kernel\",\"name\":\"DualStreamSSR/SSR8/filter8\",\"sid\":\"851\"}},\"rhs\":{\"type\":\"tile\",\"args\":[{\"type\":\"evaluable\",\"expr\":\"30\",\"value\":30},{\"type\":\"evaluable\",\"expr\":\"1\",\"value\":1}]},\"equality\":true}]"  deprecateConstraints=1
      KernelAllAttrs=|
      | s[12;12;9;9;19;14;21;23;24;21;12;24;26;26;26;27;28;9;21;23;23;23;24;25;14;19;19;29]@FunctionNameDeclFileNamePortNamesPortTypesPortSerializedTypesPortDirectionsPortWindowSizeEnablesPortWindowMarginEnablesPortSynchronicityEnablesPortSignalSizeEnablesFunctionDeclFunctionTemplateSpecKindFunctionTemplateParamNamesFunctionTemplateParamKindsFunctionTemplateParamTypesFunctionTemplateParamValuesFunctionTemplateParamEnablesClassDeclClassTemplateSpecKindClassTemplateParamNamesClassTemplateParamKindsClassTemplateParamTypesClassTemplateParamValuesClassTemplateParamEnablesClassCtorDeclsClassCtorParamNamesClassCtorParamTypesClassCtorParamSerializedTypes[1 1]@C[28 1]@t6@filtert42@../../../aie/aie_kernels/FirDoubleStream.hC[3 1]@t4@sin1t4@sin2t4@coutC[3 1]@t30@input_stream_cint16 * restrictt30@input_stream_cint16 * restrictt27@output_stream< cacc48_t > *C[3 1]@t37@{Q2{P{Tinput_stream{1{t{Scint16}}}}}}t37@{Q2{P{Tinput_stream{1{t{Scint16}}}}}}t36@{P{Toutput_stream{1{t{Scacc48_t}}}}}C[3 1]@t5@inputt5@inputt6@outputC[3 1]@l0@l0@l0@C[3 1]@l0@l0@l0@C[3 1]@l0@l0@l0@C[3 1]@l0@l0@l1@t246@namespace DoubleStream {
      | template < int NSamples, int ShiftAcc, bool DiscardSample, bool SwapRead > 
      | void FIR_MultiKernel_cout::
      | filter(input_stream_cint16 * restrict sin1, input_stream_cint16 * restrict sin2, output_stream< cacc48_t > * cout);
      | }t4@nonee[0 1]@e[0 1]@e[0 1]@e[0 1]@e[0 1]@t129@namespace DoubleStream {
      | template < int NSamples, int ShiftAcc, bool DiscardSample, bool SwapRead > class FIR_MultiKernel_cout;
      | }t8@implicitC[4 1]@t8@NSamplest8@ShiftAcct13@DiscardSamplet8@SwapReadC[4 1]@t7@nontypet7@nontypet7@nontypet7@nontypeC[4 1]@t3@intt3@intt4@boolt4@boolC[4 1]@nnnnC[4 1]@l1@l1@l1@l1@C[1 1]@t51@FIR_MultiKernel_cout(cint16 const ( & taps ) [ 4 ])C[1 1]@C[1 1]@t4@tapsC[1 1]@C[1 1]@t23@cint16 const ( &) [ 4 ]C[1 1]@C[1 1]@t20@{R{Q1{C{Scint16}4}}}
      FunctionDecl=|
      | namespace DoubleStream {
      | template < int NSamples, int ShiftAcc, bool DiscardSample, bool SwapRead > 
      | void FIR_MultiKernel_cout::
      | filter(input_stream_cint16 * restrict sin1, input_stream_cint16 * restrict sin2, output_stream< cacc48_t > * cout);
      | }
      ClassDeclTypeOptions=|
      | C[1 1]@t129@namespace DoubleStream {
      | template < int NSamples, int ShiftAcc, bool DiscardSample, bool SwapRead > class FIR_MultiKernel_cout;
      | }
      ClassDecl=|
      | namespace DoubleStream {
      | template < int NSamples, int ShiftAcc, bool DiscardSample, bool SwapRead > class FIR_MultiKernel_cout;
      | }
  filter9 : aieBasic/AIE Class Kernel  KernelAllAttrs=|  PortNames={'sin1'; 'sin2'; 'cin'; 'cout'}  PortSerializedTypes={'{Q2{P{Tinput_stream{1{t{Scint16}}}}}}'; '{Q2{P{Tinput_stream{1{t{Scint16}}}}}}'; '{P{Tinput_stream{1{t{Scacc48_t}}}}}'; '{P{Toutput_stream{1{t{Scacc48_t}}}}}'}  PortWindowSizes={0.000000000000000000e+00; 0.000000000000000000e+00; 0.000000000000000000e+00; 0.000000000000000000e+00}  PortWindowMargins={0.000000000000000000e+00; 0.000000000000000000e+00; 0.000000000000000000e+00; 0.000000000000000000e+00}  PortSynchronicities={'auto'; 'auto'; 'auto'; 'auto'}  PortSignalSizes={0.000000000000000000e+00; 0.000000000000000000e+00; 0.000000000000000000e+00; 8.000000000000000000e+00}  ClassTemplateSpecKind=implicit  ClassTemplateParamNames={'NSamples'; 'ShiftAcc'; 'DiscardSample'; 'SwapRead'}  ClassTemplateParamKinds={'nontype'; 'nontype'; 'nontype'; 'nontype'}  ClassTemplateParamTypes={'int'; 'int'; 'bool'; 'bool'}  ClassTemplateParamValues={'512', '15', '0', '0'}  ClassCtorParamNames={'taps'}  ClassCtorParamSerializedTypes={'{R{Q1{C{Scint16}4}}}'}  ClassCtorParamValues={'[-83+21i 237+54i 4086-5221i 146+91i]'}  ClassIndex=1  ClassCtorIndex=1  ClassTabVisible=on  ClassTemplateParamsVisible=on  ClassCtorDeclVisible=on  ClassCtorParamsVisible=on  FunctionTabVisible=on  FunctionDecl=|  PortAttrs={ 'input', 'sin1', 'input_stream_cint16 * restrict', '', '', '', ''; 'input', 'sin2', 'input_stream_cint16 * restrict', '', '', '', ''; 'input', 'cin', 'input_stream< cacc48_t > *', '', '', '', ''; 'output', 'cout', 'output_stream< cacc48_t > *', '', '', '', 'OUTPUT_SIZE' }  PortAttrsEnables={'off', 'off', 'off', 'off', 'off', 'off', 'off';'off', 'off', 'off', 'off', 'off', 'off', 'off';'off', 'off', 'off', 'off', 'off', 'off', 'off';'off', 'off', 'off', 'off', 'off', 'off', 'on'}  SampleTime=-1  ClassDeclTypeOptions=|  ClassDecl=|  ClassTemplateParams={ 'NSamples', 'int', 'BURST_LENGTH'; 'ShiftAcc', 'int', 'SHIFT_ACC'; 'DiscardSample', 'bool', 'FALSE'; 'SwapRead', 'bool', 'FALSE' }  ClassTemplateParamsEnables={'off', 'off', 'on';'off', 'off', 'on';'off', 'off', 'on';'off', 'off', 'on'}  ClassCtorDeclTypeOptions=C[1 1]@t54@FIR_MultiKernel_cincout(cint16 const ( & taps ) [ 4 ])  ClassCtorDecl=FIR_MultiKernel_cincout(cint16 const ( & taps ) [ 4 ])  ClassCtorParams={ 'taps', 'cint16 const ( &) [ 4 ]', 'phi_1' }  KernelHeaderFile=FirDoubleStream.h  KernelClassName=DoubleStream::FIR_MultiKernel_cincout  KernelFunction=filter  KernelSourceFile=FirDoubleStream.cpp  KernelSearchPaths={'$SRC/aie_kernels'}  PreProcOptions={}  CoreRuntimeRatio=0.9  KernelLocSpec=off  ColRowLocation=[0 0]  blockJsonConstraints="{\"type\":\"constraint\",\"constraintType\":\"coreUtilization\",\"sid\":\"852\",\"lhs\":{\"type\":\"runtimeRatio\",\"args\":{\"type\":\"kernel\",\"name\":\"DualStreamSSR_b/Subsystem/filter9\",\"sid\":\"852\"}},\"rhs\":{\"type\":\"evaluable\",\"expr\":\"0.9\",\"value\":0.9},\"equality\":true}"  deprecateConstraints=1
      KernelAllAttrs=|
      | s[12;12;9;9;19;14;21;23;24;21;12;24;26;26;26;27;28;9;21;23;23;23;24;25;14;19;19;29]@FunctionNameDeclFileNamePortNamesPortTypesPortSerializedTypesPortDirectionsPortWindowSizeEnablesPortWindowMarginEnablesPortSynchronicityEnablesPortSignalSizeEnablesFunctionDeclFunctionTemplateSpecKindFunctionTemplateParamNamesFunctionTemplateParamKindsFunctionTemplateParamTypesFunctionTemplateParamValuesFunctionTemplateParamEnablesClassDeclClassTemplateSpecKindClassTemplateParamNamesClassTemplateParamKindsClassTemplateParamTypesClassTemplateParamValuesClassTemplateParamEnablesClassCtorDeclsClassCtorParamNamesClassCtorParamTypesClassCtorParamSerializedTypes[1 1]@C[28 1]@t6@filtert42@../../../aie/aie_kernels/FirDoubleStream.hC[4 1]@t4@sin1t4@sin2t3@cint4@coutC[4 1]@t30@input_stream_cint16 * restrictt30@input_stream_cint16 * restrictt26@input_stream< cacc48_t > *t27@output_stream< cacc48_t > *C[4 1]@t37@{Q2{P{Tinput_stream{1{t{Scint16}}}}}}t37@{Q2{P{Tinput_stream{1{t{Scint16}}}}}}t35@{P{Tinput_stream{1{t{Scacc48_t}}}}}t36@{P{Toutput_stream{1{t{Scacc48_t}}}}}C[4 1]@t5@inputt5@inputt5@inputt6@outputC[4 1]@l0@l0@l0@l0@C[4 1]@l0@l0@l0@l0@C[4 1]@l0@l0@l0@l0@C[4 1]@l0@l0@l0@l1@t281@namespace DoubleStream {
      | template < int NSamples, int ShiftAcc, bool DiscardSample, bool SwapRead > 
      | void FIR_MultiKernel_cincout::
      | filter(input_stream_cint16 * restrict sin1, input_stream_cint16 * restrict sin2, input_stream< cacc48_t > * cin, output_stream< cacc48_t > * cout);
      | }t4@nonee[0 1]@e[0 1]@e[0 1]@e[0 1]@e[0 1]@t132@namespace DoubleStream {
      | template < int NSamples, int ShiftAcc, bool DiscardSample, bool SwapRead > class FIR_MultiKernel_cincout;
      | }t8@implicitC[4 1]@t8@NSamplest8@ShiftAcct13@DiscardSamplet8@SwapReadC[4 1]@t7@nontypet7@nontypet7@nontypet7@nontypeC[4 1]@t3@intt3@intt4@boolt4@boolC[4 1]@nnnnC[4 1]@l1@l1@l1@l1@C[1 1]@t54@FIR_MultiKernel_cincout(cint16 const ( & taps ) [ 4 ])C[1 1]@C[1 1]@t4@tapsC[1 1]@C[1 1]@t23@cint16 const ( &) [ 4 ]C[1 1]@C[1 1]@t20@{R{Q1{C{Scint16}4}}}
      FunctionDecl=|
      | namespace DoubleStream {
      | template < int NSamples, int ShiftAcc, bool DiscardSample, bool SwapRead > 
      | void FIR_MultiKernel_cincout::
      | filter(input_stream_cint16 * restrict sin1, input_stream_cint16 * restrict sin2, input_stream< cacc48_t > * cin, output_stream< cacc48_t > * cout);
      | }
      ClassDeclTypeOptions=|
      | C[1 1]@t132@namespace DoubleStream {
      | template < int NSamples, int ShiftAcc, bool DiscardSample, bool SwapRead > class FIR_MultiKernel_cincout;
      | }
      ClassDecl=|
      | namespace DoubleStream {
      | template < int NSamples, int ShiftAcc, bool DiscardSample, bool SwapRead > class FIR_MultiKernel_cincout;
      | }
  Phase0_out0 : Outport
  Phase0_out1 : Outport  Port=2
  Phase1_out0 : Outport  Port=3
  Phase1_out1 : Outport  Port=4
  Phase2_out0 : Outport  Port=5
  Phase2_out1 : Outport  Port=6
  Phase3_out0 : Outport  Port=7
  Phase3_out1 : Outport  Port=8
  Phase4_out0 : Outport  Port=9
  Phase4_out1 : Outport  Port=10
  Phase5_out0 : Outport  Port=11
  Phase5_out1 : Outport  Port=12
  Phase6_out0 : Outport  Port=13
  Phase6_out1 : Outport  Port=14
  Phase7_out0 : Outport  Port=15
  Phase7_out1 : Outport  Port=16
  wires:
  filter62/1 -> filter63/3
  filter1/1 -> filter2/3
  filter41/1 -> filter49/3
  filter6/1 -> filter7/3
  filter44/1 -> filter55/3
  filter17/1 -> filter24/3
  filter33/1 -> filter44/3
  filter50/1 -> filter51/3
  filter37/1 -> filter36/3
  filter36/1 -> filter35/3
  filter63/1 -> filter37/3
  filter10/1 -> filter9/3
  filter47/1 -> filter48/3
  filter52/1 -> filter53/3
  filter49/1 -> filter50/3
  filter12/1 -> filter11/3
  filter26/1 -> filter27/3
  filter25/1 -> filter26/3
  filter38/1 -> filter39/3
  filter59/1 -> filter60/3
  filter24/1 -> filter25/3
  filter32/1 -> filter33/3
  filter27/1 -> filter28/3
  filter13/1 -> filter12/3
  filter34/1 -> filter38/3
  filter19/1 -> filter18/3
  filter11/1 -> filter10/3
  filter2/1 -> filter3/3
  filter51/1 -> filter52/3
  filter40/1 -> filter41/3
  filter60/1 -> filter61/3
  filter5/1 -> filter6/3
  filter35/1 -> filter34/3
  filter45/1 -> filter43/3
  filter43/1 -> filter42/3
  filter58/1 -> filter59/3
  filter28/1 -> filter29/3
  filter18/1 -> filter22/3
  filter57/1 -> filter45/3
  filter30/1 -> filter31/3
  filter55/1 -> filter58/3
  filter53/1 -> filter54/3
  filter46/1 -> filter47/3
  filter3/1 -> filter4/3
  filter9/1 -> filter14/3
  filter14/1 -> filter15/3
  filter8/1 -> filter13/3
  filter21/1 -> filter20/3
  filter42/1 -> filter46/3
  filter16/1 -> filter17/3
  filter20/1 -> filter19/3
  filter31/1 -> filter21/3
  filter4/1 -> filter5/3
  filter56/1 -> filter57/3
  filter22/1 -> filter23/3
  filter/1 -> filter1/3
  filter48/1 -> PLIO/1
  PLIO/1 -> Phase7_out0/1
  filter48/2 -> PLIO1/1
  PLIO1/1 -> Phase7_out1/1
  filter39/1 -> PLIO2/1
  PLIO2/1 -> Phase5_out0/1
  filter39/2 -> PLIO3/1
  PLIO3/1 -> Phase5_out1/1
  filter23/1 -> PLIO4/1
  PLIO4/1 -> Phase3_out0/1
  filter23/2 -> PLIO5/1
  PLIO5/1 -> Phase3_out1/1
  filter15/1 -> PLIO6/1
  PLIO6/1 -> Phase1_out0/1
  filter15/2 -> PLIO7/1
  PLIO7/1 -> Phase1_out1/1
  P0_S0_I0/1 -> PLIO8/1
  PLIO8/1 -> filter40/1, filter32/1, filter16/1, filter/1
  P0_S1_I0/1 -> PLIO9/1
  PLIO9/1 -> filter32/2, filter40/2, filter16/2, filter/2
  P0_S0_I1/1 -> PLIO10/1
  PLIO10/1 -> filter48/1, filter39/1, filter23/1, filter15/1
  P0_S1_I1/1 -> PLIO11/1
  PLIO11/1 -> filter48/2, filter39/2, filter23/2, filter15/2
  P1_S0_I0/1 -> PLIO12/1
  PLIO12/1 -> filter41/1, filter33/1, filter17/1, filter1/1
  P1_S1_I0/1 -> PLIO13/1
  PLIO13/1 -> filter41/2, filter33/2, filter17/2, filter1/2
  P1_S0_I1/1 -> PLIO14/1
  PLIO14/1 -> filter47/1, filter38/1, filter22/1, filter14/1
  P1_S1_I1/1 -> PLIO15/1
  PLIO15/1 -> filter47/2, filter38/2, filter22/2, filter14/2
  P2_S0_I0/1 -> PLIO16/1
  PLIO16/1 -> filter44/1, filter49/1, filter24/1, filter2/1
  P2_S1_I0/1 -> PLIO17/1
  PLIO17/1 -> filter44/2, filter49/2, filter24/2, filter2/2
  P2_S0_I1/1 -> PLIO18/1
  PLIO18/1 -> filter34/1, filter46/1, filter18/1, filter9/1
  P2_S1_I1/1 -> PLIO19/1
  PLIO19/1 -> filter34/2, filter46/2, filter18/2, filter9/2
  P3_S0_I0/1 -> PLIO20/1
  PLIO20/1 -> filter55/1, filter50/1, filter25/1, filter3/1
  P3_S1_I0/1 -> PLIO21/1
  PLIO21/1 -> filter55/2, filter50/2, filter25/2, filter3/2
  P3_S0_I1/1 -> PLIO22/1
  PLIO22/1 -> filter35/1, filter42/1, filter19/1, filter10/1
  P3_S1_I1/1 -> PLIO23/1
  PLIO23/1 -> filter35/2, filter42/2, filter19/2, filter10/2
  P4_S0_I0/1 -> PLIO24/1
  PLIO24/1 -> filter58/1, filter51/1, filter26/1, filter4/1
  P4_S1_I0/1 -> PLIO25/1
  PLIO25/1 -> filter58/2, filter51/2, filter26/2, filter4/2
  P4_S0_I1/1 -> PLIO26/1
  PLIO26/1 -> filter36/1, filter43/1, filter20/1, filter11/1
  P4_S1_I1/1 -> PLIO27/1
  PLIO27/1 -> filter36/2, filter43/2, filter20/2, filter11/2
  P5_S0_I0/1 -> PLIO28/1
  PLIO28/1 -> filter52/1, filter59/1, filter27/1, filter5/1
  P5_S1_I0/1 -> PLIO29/1
  PLIO29/1 -> filter52/2, filter59/2, filter27/2, filter5/2
  P5_S0_I1/1 -> PLIO30/1
  PLIO30/1 -> filter21/1, filter37/1, filter45/1, filter12/1
  P5_S1_I1/1 -> PLIO31/1
  PLIO31/1 -> filter21/2, filter45/2, filter37/2, filter12/2
  P6_S0_I0/1 -> PLIO32/1
  PLIO32/1 -> filter60/1, filter53/1, filter28/1, filter6/1
  P6_S1_I0/1 -> PLIO33/1
  PLIO33/1 -> filter60/2, filter53/2, filter28/2, filter6/2
  P6_S0_I1/1 -> PLIO34/1
  PLIO34/1 -> filter63/1, filter57/1, filter13/1, filter31/1
  P6_S1_I1/1 -> PLIO35/1
  PLIO35/1 -> filter63/2, filter57/2, filter13/2, filter31/2
  P7_S0_I0/1 -> PLIO36/1
  PLIO36/1 -> filter54/1, filter61/1, filter29/1, filter7/1
  P7_S1_I0/1 -> PLIO37/1
  PLIO37/1 -> filter54/2, filter61/2, filter29/2, filter7/2
  P7_S0_I1/1 -> PLIO38/1
  PLIO38/1 -> filter56/1, filter62/1, filter30/1, filter8/1
  P7_S1_I1/1 -> PLIO39/1
  PLIO39/1 -> filter56/2, filter62/2, filter30/2, filter8/2
  filter7/1 -> PLIO40/1
  PLIO40/1 -> Phase0_out0/1
  filter7/2 -> PLIO41/1
  PLIO41/1 -> Phase0_out1/1
  filter29/2 -> PLIO42/1
  PLIO42/1 -> Phase2_out1/1
  filter29/1 -> PLIO43/1
  PLIO43/1 -> Phase2_out0/1
  filter61/2 -> PLIO44/1
  PLIO44/1 -> Phase4_out1/1
  filter61/1 -> PLIO45/1
  PLIO45/1 -> Phase4_out0/1
  filter54/2 -> PLIO46/1
  PLIO46/1 -> Phase6_out1/1
  filter54/1 -> PLIO47/1
  PLIO47/1 -> Phase6_out0/1
